simulink library "AEMS_Standard_Library"  (R2016b)
settings: Solver=ode45  StartTime=0.0  StopTime=10.0  RelTol=1e-3
undefined symbols (not defined in the file or in its folder): BkPY, carto, Cbx_extegr, Cbx_lpegrsys, Cbx_portegr, Cnx_bnk_nr_conf, Cnx_cyl_nr_conf, ConfigManagement, configuration_management, Cxx_dcm_io_tmr_end_xxxx, Cxx_dcm_rt_tmr_end, Cxx_DID_xxxx_IO_max, Cxx_DID_xxxx_IO_min, Cxx_egrhsofs, Cxx_vmaniegi, DEM_DEBOUNCE_FREEZE, DEM_DTR_CTL_INVISIBLE, DEM_DTR_CTL_NORMAL, Dem_DtrId2_XXX, Dem_DtrId3_XXX, Dem_DtrId4_XXX, Dem_DtrId5_XXX, Dem_DtrId6_XXX, Dem_DtrId7_XXX, Dem_DtrId8_XXX, Dem_DtrId9_XXX, Dem_DtrId_XXX, Dem_EnableConditionId2_XXX, Dem_EnableConditionId3_XXX, Dem_EnableConditionId4_XXX, Dem_EnableConditionId5_XXX, Dem_EnableConditionId6_XXX, Dem_EnableConditionId7_XXX, Dem_EnableConditionId8_XXX, Dem_EnableConditionId_XXX, Dem_EventId, Dem_EventId2_XXX, Dem_EventId3_XXX, Dem_EventId4_XXX, Dem_EventId5_XXX, Dem_EventId6_XXX, Dem_EventId7_XXX, Dem_EventId8_XXX, Dem_EventId9_XXX, Dem_EventId_Device_Faulttype, Dem_EventId_XXX, DEM_IUMPR_GENERAL_DENOMINATOR, DEM_OPCYC_IGNITION, Dem_RatioId2_XXX, Dem_RatioId3_XXX, Dem_RatioId4_XXX, Dem_RatioId5_XXX, Dem_RatioId6_XXX, Dem_RatioId7_XXX, Dem_RatioId8_XXX, Dem_RatioId_XXX, Dem_StorageConditionId2_XXX, Dem_StorageConditionId3_XXX, Dem_StorageConditionId4_XXX, Dem_StorageConditionId5_XXX ... (+65)
libraries: AEMS_Standard_Library x477, simulink x2
(part 3 of 39)

== system AEMS_Standard_Library/DCM ==
  note: AUTOSAR INTERFACE for DCM TO BE USED IN
      | DataServices or RoutineServices_DIDAbstract_AUTOSAR_Interface
  note: Applicative DCM:
      | To be used in functional specifications
  note: Supplier API Call:
      | To be used to call Supplier API
  AEMS_API_SUPPLIER_CALL : Subsystem  Tag=[LIB]  mask(AEMS_API_SUPPLIER_CALL){portName=port, operationPrototype=API_Supplier_Fcn(IN uint8 In1[12], IN int16 In2[3], OUT single Out1[1]), NumInputs=2, NumOutputs=1, API_Name=Ex_API, Ptr_Arg=01}
      mask prompts: portName "Client Port name"; operationPrototype "API Supplier Function Call Name"; NumInputs "Number of Inputs"; NumOutputs "Number of Outputs"; Ptr_Arg "Pointer_Arguments"
      mask help:
      | This block is used to call the function prototype specified as "Supplier_API_name" in the generated C-code with
      | arguments provided as inputs.
      |
      | Example Supplier API Call:
      | API_Supplier_Fcn(IN uint8 In1[12], IN int16 In2[3], OUT single Out1[1]);
      |
      | Code expected:
      | API_Supplier_Fcn(In1,In2,&Out1)
      mask init:
      | BlkName = gcb;
      | hblk = gcbh;
      | 
      | % if strcmp(get_param(hblk,'LinkStatus'),'resolved')
      | %     set_param(hblk,'LinkStatus','inactive');
      | % else
      | %     %already disabled or none
      | % end
      | datatypelist={'uint8','int8','uint16','int16','uint32','int32','boolean','single','double'};
      | 
      | ProtoTypeStr = get_param(hblk,'operationPrototype');
      | 
      | % try 
      | flag_err = 0;
      | st = regexp(ProtoTypeStr,'(');
      | et = regexp(ProtoTypeStr,')');
      | if isempty(st) || isempty(et)
      |     flag_err = 1;
      |     error('OperationPrototype must contain braces ''('' and '')''');
      | elseif length(st)>1 || length(et)>1
      |     flag_err = 1;
      |     error('Invalid format for  Operation Prototype');
      | else
      |     API_Name = ProtoTypeStr(1:(st-1));
      |     Proto_str = regexprep(ProtoTypeStr,[API_Name,'|',')|('],'');
      |     
      |     %     Proto_str = regexprep(regexprep(ProtoTypeStr,API_Name,''),')|(',''); % alternative
      |     
      |     NumInputs = length(regexp(ProtoTypeStr,'IN |INOUT '));
      |     NumOutputs = length(regexp(ProtoTypeStr,'[^IN]OUT '));
      |     
      |     if NumInputs ~= 0 || NumOutputs ~= 0
      |         parts= regexp(strtrim(regexp(strtrim(Proto_str),',','split')),' ' ,'split');
      |     else
      |         parts ='';
      |     end
      |     for i=1:numel(parts)
      |         if numel(parts{i})~=3
      |             flag_err = 1;
      |             error('Invalid format:Avoid extra spaces in between Argument literals (Ex: IN single In1)');
      |         end
      |     end
      | end
      | 
      | inporthdl = find_system(BlkName,'FollowLinks','on','LookunderMasks','all','regexp','on','BlockType','Inport');
      | outporthdl = find_system(BlkName,'FollowLinks','on','LookunderMasks','all','regexp','on','BlockType','Outport');
      | 
      | isChanged=0; 
      | for i=1:numel(parts) 
      |     if ~isempty(regexp(parts{i}{1},'IN|OUT|INOUT','once'))
      |         if ismember(parts{i}{2},datatypelist) || isempty(parts{i}{2})
      |             tmp_DT = parts{i}{2};
      |         else
      |             error(['Datatype ''' parts{i}{2} ''' is invalid']);
      |         end
      |         if length(regexp(parts{i}{3},'['))==1 && length(regexp(parts{i}{3},']'))==1
      |             % dimension specified
      |         elseif isempty(regexp(parts{i}{3},'[')) && isempty(regexp(parts{i}{3},']'))
      |             % dimension not specified
      |         else
      |             error('Avoid Extra/unexpected braces (''['' and '']'').Enter Correct Format(Ex IN uint8 a[12])');
      |         end
      |         [Port_name,Port_Dim] = strtok(parts{i}{3},'[');
      |         if ~isempty(regexp(Port_name,'^\d|^_','once'))
      |             error(sprintf(['Invalid Inport/Outport name:' Port_name '\nName should start with an alphabet']));
      |         elseif ~isempty(regexp(Port_name,'_$','once'))
      |             error(sprintf(['Invalid Inport/Outport name:' Port_name '\nName shouldn''t end with underscore(_)']));
      |         else
      | 
      |             if isempty(regexp(Port_Dim,'([\d+\])','once'))
      |                 error('Incorrect Dimension entered.Check and Enter Correct Format(Ex IN uint8 a[12])');
      |             else
      |                 tmp_Dim = strtok(Port_Dim,'^[]$');
      |             end
      | 
      |             if isempty(regexp(Port_name,'\W','once'))
      |                 tmp_Name = Port_name;
      |             else
      |                 error('Special characters otherthan underscore( _ ) are not allowed in Port names');
      |             end
      |         end
      |     end
      |     if strcmp(parts{i}{1},'IN') || strcmp(parts{i}{1},'INOUT')
      |         %         NumInputs = NumInputs+1;
      |         In_InOut_Names = tmp_Name;
      |         In_InOut_Types = tmp_DT;
      |         In_InOut_Dim = tmp_Dim;
      |         inporthdl = find_system(hblk,'FollowLinks','on','LookunderMasks','all','regexp','on','BlockType','Inport','Name',In_InOut_Names);
      |         if isempty(inporthdl)
      |            isChanged=1; 
      |            break;
      |         else
      |            datatype=get_param(inporthdl,'OutDataTypeStr'); 
      |            indim=get_param(inporthdl,'PortDimensions');
      |            if ~isequal(datatype,In_InOut_Types)||~isequal(indim,In_InOut_Dim)
      |               isChanged=1; 
      |               break;               
      |            end
      |         end
      |     elseif strcmp(parts{i}{1},'OUT')
      |         %         NumOutputs = NumOutputs+1;
      |         Out_Names = tmp_Name;
      |         Out_Types = tmp_DT;
      |         Out_Dim = tmp_Dim;
      |         outporthdl = find_system(hblk,'FollowLinks','on','LookunderMasks','all','regexp','on','BlockType','Outport','Name',Out_Names);
      |         if isempty(outporthdl)
      |            isChanged=1; 
      |            break;
      |         else
      |            datatype=get_param(outporthdl,'OutDataTypeStr'); 
      |            indim=get_param(outporthdl,'PortDimensions');
      |            if ~isequal(datatype,Out_Types)||~isequal(indim,Out_Dim)
      |               isChanged=1; 
      |               break;               
      |            end
      |         end        
      |         
      |     else
      |         error('Direction must be IN, INOUT or OUT');
      |     end
      | end      
      | % if length(st)~=length(et) && flag_err_occur==0
      | %     flag_err = 1;
      | %     errordlg('Invalid format for  Operation Prototype');
      | % end
      | 
      | % if evalin('base','flag_err')==0
      | if flag_err == 0&&isChanged
      |     % To Remove Lines and Terminator/Ground
      |     lines = find_system(hblk,'LookUnderMasks','all','FollowLinks','On','FindAll','on','Type','line');
      |     GndTer = find_system(hblk,'LookUnderMasks','all','FollowLinks','On','regexp','On','FindAll','on','BlockType','^Ground$|^Terminator$|^DataTypeConversion$');
      | %     GndTer = find_system(hblk,'LookUnderMasks','all','FollowLinks','On','regexp','On','FindAll','on','BlockType','^Ground$|^Terminator$');
      |     tobe_del = [lines;GndTer];
      |     for i=1:length(tobe_del)
      |         try
      |             delete_line(tobe_del(i));
      |         catch
      |             delete_block(tobe_del(i));
      |         end
      |     end
      |     
      |     In_InOut_Names = {};
      |     In_InOut_Types = {};
      |     In_InOut_Dim = {};
      |     Out_Names = {};
      |     Out_Types = {};
      |     Out_Dim = {};
      |     % NumOutputs = 0;
      |     % NumInputs = 0;
      |     % parts = evalin('base','parts');
      |     for i=1:numel(parts)
      |         if ~isempty(regexp(parts{i}{1},'IN|OUT|INOUT','once'))
      |             if ismember(parts{i}{2},datatypelist) || isempty(parts{i}{2})
      |                 tmp_DT = parts{i}{2};
      |             else
      |                 error(['Datatype ''' parts{i}{2} ''' is invalid']);
      |             end
      |             if length(regexp(parts{i}{3},'['))==1 && length(regexp(parts{i}{3},']'))==1
      |                 % dimension specified
      |             elseif isempty(regexp(parts{i}{3},'[')) && isempty(regexp(parts{i}{3},']'))
      |                 % dimension not specified
      |             else
      |                 error('Avoid Extra/unexpected braces (''['' and '']'').Enter Correct Format(Ex IN uint8 a[12])');
      |             end
      |             [Port_name,Port_Dim] = strtok(parts{i}{3},'[');
      |             if ~isempty(regexp(Port_name,'^\d|^_','once'))
      |                 error(sprintf(['Invalid Inport/Outport name:' Port_name '\nName should start with an alphabet']));
      |             elseif ~isempty(regexp(Port_name,'_$','once'))
      |                 error(sprintf(['Invalid Inport/Outport name:' Port_name '\nName shouldn''t end with underscore(_)']));
      |             else
      |                 
      |                 if isempty(regexp(Port_Dim,'([\d+\])','once'))
      |                     error('Incorrect Dimension entered.Check and Enter Correct Format(Ex IN uint8 a[12])');
      |                 else
      |                     tmp_Dim = strtok(Port_Dim,'^[]$');
      |                 end
      |                 
      |                 if isempty(regexp(Port_name,'\W','once'))
      |                     tmp_Name = Port_name;
      |                 else
      |                     error('Special characters otherthan underscore( _ ) are not allowed in Port names');
      |                 end
      |             end
      |         end
      |         if strcmp(parts{i}{1},'IN') || strcmp(parts{i}{1},'INOUT')
      |             %         NumInputs = NumInputs+1;
      |             In_InOut_Names = [In_InOut_Names,tmp_Name];
      |             In_InOut_Types = [In_InOut_Types,tmp_DT];
      |             In_InOut_Dim = [In_InOut_Dim,tmp_Dim];
      |         elseif strcmp(parts{i}{1},'OUT')
      |             %         NumOutputs = NumOutputs+1;
      |             Out_Names = [Out_Names,tmp_Name];
      |             Out_Types = [Out_Types,tmp_DT];
      |             Out_Dim = [Out_Dim,tmp_Dim];
      |         else
      |             error('Direction must be IN, INOUT or OUT');
      |         end
      |     end
      |     
      |     %To delete unwanted Inport/Outport blocks
      |     Inports_exist = get_param(find_system(BlkName,'LookUnderMasks','All','FollowLinks','On','regexp','On','BlockType','Inport'),'Name');
      |     Outports_exist = get_param(find_system(BlkName,'LookUnderMasks','All','FollowLinks','On','regexp','On','BlockType','Outport'),'Name');
      |     Inports_to_be_del = setdiff(Inports_exist,In_InOut_Names);
      |     Outports_to_be_del = setdiff(Outports_exist,Out_Names);
      |     ports_to_be_del = [Inports_to_be_del;Outports_to_be_del];
      |     for n=1:numel(ports_to_be_del)
      |         delete_block([BlkName,'/',ports_to_be_del{n}]);
      |     end
      |     
      |     tmp_in_out_names = [In_InOut_Names,Out_Names];
      |     
      |     if ~isequal(length(unique(tmp_in_out_names)),length(tmp_in_out_names))
      |         error('Port names must be unique')
      |     else
      |         %To add In Ports
      |         % NumInputs = numel(IN_OR_INOUT_Strings);
      |         for n=1:NumInputs
      |             Pos_Y1 = (10+((n-1)*40));
      |             Blk_Pos = [20,Pos_Y1,50,Pos_Y1+15];
      |             Term_Pos = [115,Pos_Y1,135,Pos_Y1+20];
      |             try
      |                 add_block('built-in/Inport',[BlkName,'/',In_InOut_Names{n}]);
      |             catch
      |                 set_param([BlkName,'/',In_InOut_Names{n}],'Port',num2str(n));
      |             end
      |             set_param([BlkName,'/',In_InOut_Names{n}],...
      |                 'Position',Blk_Pos,...
      |                 'OutDataTypeStr',In_InOut_Types{n},...
      |                 'PortDimensions',In_InOut_Dim{n},...
      |                 'Backgroundcolor','green');
      |             add_block('built-in/Terminator',[BlkName,'/T_',In_InOut_Names{n}],'Position',Term_Pos,'ShowName','off');
      |             add_line(BlkName,[In_InOut_Names{n},'/1'],['T_',In_InOut_Names{n},'/1']);
      |         end
      |         
      |         %To add Out Ports
      |         for n=1:NumOutputs
      |             Pos_Y1 = (10+((n-1)*40));
      |             Blk_Pos = [400,Pos_Y1,430,Pos_Y1+15];
      |             Con_Pos = [300,Pos_Y1,330,Pos_Y1+20];
      |             Gnd_Pos = [210,Pos_Y1,230,Pos_Y1+20];
      |             try
      |                 add_block('built-in/Outport',[BlkName,'/',Out_Names{n}],'Position',Blk_Pos,'OutDataTypeStr',Out_Types{n},'Backgroundcolor','orange');
      |             catch
      |                 set_param([BlkName,'/',Out_Names{n}],'Port',num2str(n),'Position',Blk_Pos,'OutDataTypeStr',Out_Types{n},'Backgroundcolor','orange');
      |             end
      |             set_param([BlkName,'/',Out_Names{n}],...
      |                 'Position',Blk_Pos,...
      |                 'OutDataTypeStr',Out_Types{n},...
      |                 'PortDimensions',Out_Dim{n},...
      |                 'Backgroundcolor','orange');
      |             add_block('built-in/Ground',[BlkName,'/G_',Out_Names{n}],'Position',Gnd_Pos,'ShowName','off');
      |             add_block('built-in/DatatypeConversion',[BlkName,'/Conv_',Out_Names{n}],'Position',Con_Pos,'ShowName','off');
      |             add_line(BlkName,['Conv_',Out_Names{n},'/1'],[Out_Names{n},'/1']);
      |             add_line(BlkName,['G_',Out_Names{n},'/1'],['Conv_',Out_Names{n},'/1']);
      |         end
      |         mask_data = Simulink.Mask.get(hblk);
      |         mask_data.IconOpaque = 'off';
      |         set_param(hblk,...
      |             'NumInputs',num2str(NumInputs),...
      |             'NumOutputs',num2str(NumOutputs));
      |     end
      | end
      | 
      | % catch ErrorException
      | %     Message = sprintf('Message : %s', ErrorException.message);
      | %     for ie=1:length(ErrorException.stack)
      | %         Message = sprintf('%s\nFilename : %s', Message, ErrorException.stack(ie).file);
      | %         Message = sprintf('%s\nName : %s', Message, ErrorException.stack(ie).name);
      | %         Message = sprintf('%s\nLine : %i', Message, ErrorException.stack(ie).line);
      | %     end
      | %     disp(Message);    
      | % end
      settings: AttributesFormatString="%<MaskType>\\nPrototype: %<operationPrototype>\\nNo. of Inputs :%<NumInputs>  No of Outputs: %<NumOutputs>"
      mask Display: disp('AEMS_API_SUPPLIER_CALL');
  AEMS_APP_DID_WRITEDATA : Subsystem  Tag=[LIB]  mask(AEMS_APP_DID_WRITEDATA){}
      mask help:
      | Gets the output for DID variable depends on request write from tools. If Request write comes from DCM tools, DID variable get value from DCM tools if not it gets value from strategy’s calculation.
      |
      | -INPUTS-
      | Value_DID_Write: DID value from DCM Tools
      | Request_Write_DID: Request Write from DCM Tools
      | Strategy: Value calculated from strategy
      |
      | -OUTPUTS-
      | DID_Var: Value DID for output
      settings: AttributesFormatString=%<MaskType>
      mask Help:
      | eval('path_lib=fileparts(which(''AEMS_Standard_Library''));');
      | mskblk=get_param(gcbh,'MaskType');
      | doc_path = [path_lib '\Help\',mskblk,'.pdf'];
      | eval('open(doc_path)');
  AEMS_APP_REQUEST_IOCONTROL : Subsystem  Tag=[LIB]  mask(AEMS_APP_REQUEST_IOCONTROL){DIDAbstract=DCM_IO_XXXX, Cxx_dcm_io_tmr_end_xxxx=Cxx_dcm_io_tmr_end_xxxx}
      mask prompts: DIDAbstract "DID Abstract"; Cxx_dcm_io_tmr_end_xxxx "Duration of Timer (in milisecond)"
      mask help:
      | IO request is activated by Request from ShortTermAdjustment under the control of
      | Request from ReturnControlToECU status, Generic Condition, Specific condition and Timer End of XXXX DID Abstract.
      | Output value of DID XXXX from Callback ShorttermAdjustment.
      |
      | -INPUTS-
      | Req_stadj_stt_xxxx: Request from ShortTermAdjustment status of XXXX
      | Req_rcecu_stt_xxxx: Request from ReturnControlToECU status of XXXX
      | Generic_Condition: Generic condition
      | Specific_Condition_xxxx: Specific condition of XXXX DID
      | Value_Write_stadj_xxxx: Value of IO Signal DID XXX from ShortTermAdjustment
      |
      | -OUTPUTS-
      | Flag_io_request_xxxx: Output of IO request controlled
      | Flag_dcm_io_tmr_end_xxxx: Timer End Status of XXXX
      | Dcm_io_tmr_xxxx: Timer which counts down from value defined in Duration of Timer in miliseconde
      | Val_io_request_xxxx: Output of IO Signal DID XXX from ShortTermAdjustment
      |
      | -PARAMETERS-
      | DID Abstract: Abstract of DID
      | Duration of Timer: Duration of Timer
      mask init:
      | hh = gcbh;
      | DIDAbstractstr=get_param(hh,'DIDAbstract'); 
      | namepi1=strcat('Req_stadj_',DIDAbstractstr);
      | namepi2=strcat('Req_rcecu_',DIDAbstractstr);
      | namepi3='Generic_Condition';
      | namepi4=strcat('Specific_Condition_',DIDAbstractstr);
      | namepi5=strcat('Value_Write_stadj_',DIDAbstractstr);
      | % namepi5='Req_tmr_end_xxxx';
      | namepo1=strcat('Flag_io_request_',DIDAbstractstr);
      | namepo2=strcat('Flag_dcm_io_tmr_end_',DIDAbstractstr);
      | namepo3=strcat('Dcm_io_tmr_',DIDAbstractstr);
      | namepo4=strcat('Val_io_request_',DIDAbstractstr);
      | 
      | % encond_b1 = find_system(gcb,'LookUnderMasks','all','FollowLinks','on','Name','Cxx_dcm_io_tmr_end_xxxx');
      | % set_param([encond_b1{:}],'Value',char(Cxx_dcm_io_tmr_end_xxxx));
      settings: AttributesFormatString=|
      | %<MaskType>
      | DID Abstract : %<DIDAbstract>
      | Duration of Timer : %<Cxx_dcm_io_tmr_end_xxxx>
      mask Help:
      | eval('path_lib=fileparts(which(''AEMS_Standard_Library''));');
      | mskblk=get_param(gcbh,'MaskType');
      | doc_path = [path_lib '\Help\',mskblk,'.pdf'];
      | eval('open(doc_path)');
      mask Display:
      | port_label('input',1,namepi1);
      | port_label('input',2,namepi2);
      | port_label('input',3,namepi3);
      | port_label('input',4,namepi4);
      | port_label('input',5,namepi5);
      | port_label('output',1,namepo1);
      | port_label('output',2,namepo2);
      | port_label('output',3,namepo3);
      | port_label('output',4,namepo4);
  AEMS_APP_REQUEST_ROUTINE : Subsystem  Tag=[LIB]  mask(AEMS_APP_REQUEST_ROUTINE){DIDAbstract=DCM_RT_XXXX, Cxx_dcm_rt_tmr_end=Cxx_dcm_rt_tmr_end}
      mask prompts: DIDAbstract "RID Abstract"; Cxx_dcm_rt_tmr_end "Duration of Timer (in second)"
      mask help:
      | Retrun flags of START Callback STOP Callback from DCM.
      | Flag START is enabled if there is a change from Request of START Callback
      | Flag STOP is activated by Request from STOP Callback, Generic Condition, Specific condition and Timer End of XXXX RID Abstract.
      |
      | -INPUTS-
      | Req_sta_stt_xxxx: Request from START status of XXXX
      | Req_stop_stt_xxxx: Request from STOP status of XXXX
      | Generic_Condition: Generic condition
      | Specific_Condition_xxxx: Specific condition of XXXX RID during Routine Callback
      |
      | -OUTPUTS-
      | Flag_sta_xxxx: Output of request from START Callback
      | Flag_stop_xxxx: Output of request from STOP Callback
      | Flag_dcm_rt_tmr_end: Timer End Status
      | Dcm_rt_tmr_xxxx: Timer which counts down from value defined in Duration of Timer in seconde
      |
      | -PARAMETERS-
      | RID Abstract: Abstract of RID
      | Duration of Timer: Duration of Timer
      mask init:
      | hh = gcbh;
      | DIDAbstractstr=get_param(hh,'DIDAbstract'); 
      | namepi1=strcat('Req_sta_',DIDAbstractstr);
      | namepi2=strcat('Req_stop_',DIDAbstractstr);
      | namepi3='Generic_Condition';
      | namepi4=strcat('Specific_Condition_',DIDAbstractstr);
      | % namepi5='Req_tmr_end';
      | namepo1=strcat('Flag_sta_',DIDAbstractstr);
      | namepo2=strcat('Flag_stop_',DIDAbstractstr);
      | namepo3=strcat('Flag_dcm_rt_tmr_end_',DIDAbstractstr);
      | namepo4=strcat('Dcm_rt_tmr_',DIDAbstractstr);
      settings: AttributesFormatString=|
      | %<MaskType>
      | RID Abstract : %<DIDAbstract>
      | Duration of Timer : %<Cxx_dcm_rt_tmr_end>
      mask Help:
      | eval('path_lib=fileparts(which(''AEMS_Standard_Library''));');
      | mskblk=get_param(gcbh,'MaskType');
      | doc_path = [path_lib '\Help\',mskblk,'.pdf'];
      | eval('open(doc_path)');
      mask Display:
      | port_label('input',1,namepi1);
      | port_label('input',2,namepi2);
      | port_label('input',3,namepi3);
      | port_label('input',4,namepi4);
      | port_label('output',1,namepo1);
      | port_label('output',2,namepo2);
      | port_label('output',3,namepo3);
      | port_label('output',4,namepo4);
  AEMS_DCM_CLEARDIAGNOSTICINFORMATION : Subsystem  Tag=[LIB]  mask(AEMS_DCM_CLEARDIAGNOSTICINFORMATION){}
      mask help:
      | This library calls AUTOSAR standard functions.
      | To know more details, please refer AUTOSAR [SWS_Dem_00241].
      settings: AttributesFormatString=%<MaskType>
      mask Display: disp(['Dcm_ClearDiagnosticInformation']);
  AEMS_DCM_CONDITIONCHECKREAD : Subsystem  Tag=[LIB]  mask(AEMS_DCM_CONDITIONCHECKREAD){DIDAbstract=DCM_DID_XXXX}
      mask prompts: DIDAbstract "DID Abstract"
      mask help:
      | This function requests to the application to start the execution of a routine.
      | AUTOSAR Interface: Xxx_Start (Ref. [SWS_Dcm_01203])
      |
      | Std_ReturnType Xxx_ConditionCheckRead(Dcm_NegativeResponseCodeType* ErrorCode)
      |
      | ErrorCode: terminated to represent return values to DCM Tools.
      |
      | -INPUTS-
      | Condition_checkread: Condition check read
      |
      | -PARAMETERS-
      | DID Abstract: Abstract of DID
      mask init:
      | hh = gcbh;
      | DIDAbstractstr=get_param(hh,'DIDAbstract'); 
      | Callbkstr=strcat('DataServices_',strtrim(DIDAbstractstr),'_WriteData');
      | namepi1='Generic_Conditions_Routine';
      | namepi2=strcat('Specific_Conditions_Routine_',DIDAbstractstr);
      | namepi3='Routine_Status';
      | namepi4=strcat('Routine_Status_',DIDAbstractstr);
      | namepo1=strcat('Flag_Request_',DIDAbstractstr);
      settings: AttributesFormatString=|
      | %<MaskType>
      | DID Abstract: %<DIDAbstract>
      mask Help:
      | eval('path_lib=fileparts(which(''AEMS_Standard_Library''));');
      | mskblk=get_param(gcbh,'MaskType');
      | doc_path = [path_lib '\Help\',mskblk,'.pdf'];
      | eval('open(doc_path)');
      mask Display:
      | % port_label('input',1,namepi1);
      | % port_label('input',2,namepi2);
      | % port_label('input',3,namepi3);
      | % port_label('input',4,namepi4);
      | % port_label('output',1,namepo1);
  AEMS_DCM_DID_READDATA : Subsystem  Tag=[LIB]  mask(AEMS_DCM_DID_READDATA){DIDAbstract=DCM_DID_XXXX, NumDIDVar=1, RaDIDVar1=[0,255], OffsetDIDVar1=0, ResolDIDVar1=1, DataTypeDIDVar1=uint8, In_DID_Name_1=Val_did_1, RaDIDVar2=[-128,127], OffsetDIDVar2=0, ResolDIDVar2=1, DataTypeDIDVar2=int8, In_DID_Name_2=Val_did_2, RaDIDVar3=[0,1], OffsetDIDVar3=0, ResolDIDVar3=1, DataTypeDIDVar3=int16, In_DID_Name_3=Val_did_3, RaDIDVar4=[0,100], OffsetDIDVar4=0, ResolDIDVar4=1, DataTypeDIDVar4=uint8, In_DID_Name_4=Val_did_4, RaDIDVar5=[0,1], OffsetDIDVar5=0, ResolDIDVar5=1, DataTypeDIDVar5=uint16, In_DID_Name_5=Val_did_5, RaDIDVar6=[0,1], OffsetDIDVar6=0, ResolDIDVar6=1, DataTypeDIDVar6=uint8, In_DID_Name_6=Val_did_6, RaDIDVar7=[0,1], OffsetDIDVar7=0, ResolDIDVar7=1, DataTypeDIDVar7=uint8, In_DID_Name_7=Val_did_7, RaDIDVar8=[0,1], OffsetDIDVar8=0, ResolDIDVar8=1, DataTypeDIDVar8=uint8, In_DID_Name_8=Val_did_8, RaDIDVar9=[0,1], OffsetDIDVar9=0, ResolDIDVar9=1, DataTypeDIDVar9=uint8, In_DID_Name_9=Val_did_9, RaDIDVar10=[0,1], OffsetDIDVar10=0, ResolDIDVar10=1, DataTypeDIDVar10=uint8, In_DID_Name_10=Val_did_10, RaDIDVar11=[0,1], OffsetDIDVar11=0, ResolDIDVar11=1, DataTypeDIDVar11=uint8, In_DID_Name_11=Val_did_11, RaDIDVar12=[0,1], OffsetDIDVar12=0, ResolDIDVar12=1, DataTypeDIDVar12=uint8, In_DID_Name_12=Val_did_12, RaDIDVar13=[0,1], OffsetDIDVar13=0, ResolDIDVar13=1, DataTypeDIDVar13=uint8, In_DID_Name_13=Val_did_13, RaDIDVar14=[0,1], OffsetDIDVar14=0, ResolDIDVar14=1, DataTypeDIDVar14=uint8, In_DID_Name_14=Val_did_14, RaDIDVar15=[0,1], OffsetDIDVar15=0, ResolDIDVar15=1, DataTypeDIDVar15=uint8, In_DID_Name_15=Val_did_15, RaDIDVar16=[0,1], OffsetDIDVar16=0, ResolDIDVar16=1, DataTypeDIDVar16=uint8, In_DID_Name_16=Val_did_16, RaDIDVar17=[0,1], OffsetDIDVar17=0, ResolDIDVar17=1, DataTypeDIDVar17=uint8, In_DID_Name_17=Val_did_17, RaDIDVar18=[0,1], OffsetDIDVar18=0, ResolDIDVar18=1, DataTypeDIDVar18=uint8, In_DID_Name_18=Val_did_18, RaDIDVar19=[0,1], OffsetDIDVar19=0, ResolDIDVar19=1, DataTypeDIDVar19=uint8, In_DID_Name_19=Val_did_19, RaDIDVar20=[0,1], OffsetDIDVar20=0, ResolDIDVar20=1, DataTypeDIDVar20=uint8, In_DID_Name_20=Val_did_20, RaDIDVar21=[0,1], OffsetDIDVar21=0, ResolDIDVar21=1, DataTypeDIDVar21=uint8, In_DID_Name_21=Val_did_21, RaDIDVar22=[0,1], OffsetDIDVar22=0, ResolDIDVar22=1, DataTypeDIDVar22=uint8, In_DID_Name_22=Val_did_22, RaDIDVar23=[0,1], OffsetDIDVar23=0, ResolDIDVar23=1, DataTypeDIDVar23=uint8, In_DID_Name_23=Val_did_23, RaDIDVar24=[0,1], OffsetDIDVar24=0, ResolDIDVar24=1, DataTypeDIDVar24=uint8, In_DID_Name_24=Val_did_24, RaDIDVar25=[0,1], OffsetDIDVar25=0, ResolDIDVar25=1, DataTypeDIDVar25=uint8, In_DID_Name_25=Val_did_25, RaDIDVar26=[0,1], OffsetDIDVar26=0, ResolDIDVar26=1, DataTypeDIDVar26=uint8, In_DID_Name_26=Val_did_26, RaDIDVar27=[0,1], OffsetDIDVar27=0, ResolDIDVar27=1, DataTypeDIDVar27=uint8, In_DID_Name_27=Val_did_27, RaDIDVar28=[0,1], OffsetDIDVar28=0, ResolDIDVar28=1, DataTypeDIDVar28=uint8, In_DID_Name_28=Val_did_28, RaDIDVar29=[0,1], OffsetDIDVar29=0, ResolDIDVar29=1, DataTypeDIDVar29=uint8, In_DID_Name_29=Val_did_29, RaDIDVar30=[0,1], OffsetDIDVar30=0, ResolDIDVar30=1, DataTypeDIDVar30=uint8, In_DID_Name_30=Val_did_30, RaDIDVar31=[0,1], OffsetDIDVar31=0, ResolDIDVar31=1, DataTypeDIDVar31=uint8, In_DID_Name_31=Val_did_31, RaDIDVar32=[0,1], OffsetDIDVar32=0, ResolDIDVar32=1, DataTypeDIDVar32=uint8, In_DID_Name_32=Val_did_32, RaDIDVar33=[0,1], OffsetDIDVar33=0, ResolDIDVar33=1, DataTypeDIDVar33=uint8, In_DID_Name_33=Val_did_33, RaDIDVar34=[0,1], OffsetDIDVar34=0, ResolDIDVar34=1, DataTypeDIDVar34=uint8, In_DID_Name_34=Val_did_34, RaDIDVar35=[0,1], OffsetDIDVar35=0, ResolDIDVar35=1, DataTypeDIDVar35=uint8, In_DID_Name_35=Val_did_35, RaDIDVar36=[0,1], OffsetDIDVar36=0, ResolDIDVar36=1, DataTypeDIDVar36=uint8, In_DID_Name_36=Val_did_36, RaDIDVar37=[0,1], OffsetDIDVar37=0, ResolDIDVar37=1, DataTypeDIDVar37=uint8, In_DID_Name_37=Val_did_37, RaDIDVar38=[0,1], OffsetDIDVar38=0, ResolDIDVar38=1, DataTypeDIDVar38=uint8, In_DID_Name_38=Val_did_38, RaDIDVar39=[0,1], OffsetDIDVar39=0, ResolDIDVar39=1, DataTypeDIDVar39=uint8, In_DID_Name_39=Val_did_39, RaDIDVar40=[0,1], OffsetDIDVar40=0, ResolDIDVar40=1, DataTypeDIDVar40=uint8, In_DID_Name_40=Val_did_40, RaDIDVar41=[0,1], OffsetDIDVar41=0, ResolDIDVar41=1, DataTypeDIDVar41=uint8, In_DID_Name_41=Val_did_41, RaDIDVar42=[0,1], OffsetDIDVar42=0, ResolDIDVar42=1, DataTypeDIDVar42=uint8, In_DID_Name_42=Val_did_42, RaDIDVar43=[0,1], OffsetDIDVar43=0, ResolDIDVar43=1, DataTypeDIDVar43=uint8, In_DID_Name_43=Val_did_43, RaDIDVar44=[0,1], OffsetDIDVar44=0, ResolDIDVar44=1, DataTypeDIDVar44=uint8, In_DID_Name_44=Val_did_44, RaDIDVar45=[0,1], OffsetDIDVar45=0, ResolDIDVar45=1, DataTypeDIDVar45=uint8, In_DID_Name_45=Val_did_45, RaDIDVar46=[0,1], OffsetDIDVar46=0, ResolDIDVar46=1, DataTypeDIDVar46=uint8, In_DID_Name_46=Val_did_46, RaDIDVar47=[0,1], OffsetDIDVar47=0, ResolDIDVar47=1, DataTypeDIDVar47=uint8, In_DID_Name_47=Val_did_47, RaDIDVar48=[0,1], OffsetDIDVar48=0, ResolDIDVar48=1, DataTypeDIDVar48=uint8, In_DID_Name_48=Val_did_48, RaDIDVar49=[0,1], OffsetDIDVar49=0, ResolDIDVar49=1, DataTypeDIDVar49=uint8, In_DID_Name_49=Val_did_49, RaDIDVar50=[0,1], OffsetDIDVar50=0, ResolDIDVar50=1, DataTypeDIDVar50=uint8, In_DID_Name_50=Val_did_50, RaDIDVar51=[0,1], OffsetDIDVar51=0, ResolDIDVar51=1, DataTypeDIDVar51=uint8, In_DID_Name_51=Val_did_51, RaDIDVar52=[0,1], OffsetDIDVar52=0, ResolDIDVar52=1, DataTypeDIDVar52=uint8, In_DID_Name_52=Val_did_52, RaDIDVar53=[0,1], OffsetDIDVar53=0, ResolDIDVar53=1, DataTypeDIDVar53=uint8, In_DID_Name_53=Val_did_53, RaDIDVar54=[0,1], OffsetDIDVar54=0, ResolDIDVar54=1, DataTypeDIDVar54=uint8, In_DID_Name_54=Val_did_54, RaDIDVar55=[0,1], OffsetDIDVar55=0, ResolDIDVar55=1, DataTypeDIDVar55=uint8, In_DID_Name_55=Val_did_55, RaDIDVar56=[0,1], OffsetDIDVar56=0, ResolDIDVar56=1, DataTypeDIDVar56=uint8, In_DID_Name_56=Val_did_56, RaDIDVar57=[0,1], OffsetDIDVar57=0, ResolDIDVar57=1, DataTypeDIDVar57=uint8, In_DID_Name_57=Val_did_57, RaDIDVar58=[0,1], OffsetDIDVar58=0, ResolDIDVar58=1, DataTypeDIDVar58=uint8, In_DID_Name_58=Val_did_58, RaDIDVar59=[0,1], OffsetDIDVar59=0, ResolDIDVar59=1, DataTypeDIDVar59=uint8, In_DID_Name_59=Val_did_59, RaDIDVar60=[0,1], OffsetDIDVar60=0, ResolDIDVar60=1, DataTypeDIDVar60=uint8, In_DID_Name_60=Val_did_60, RaDIDVar61=[0,1], OffsetDIDVar61=0, ResolDIDVar61=1, DataTypeDIDVar61=uint8, In_DID_Name_61=Val_did_61, RaDIDVar62=[0,1], OffsetDIDVar62=0, ResolDIDVar62=1, DataTypeDIDVar62=uint8, In_DID_Name_62=Val_did_62, RaDIDVar63=[0,1], OffsetDIDVar63=0, ResolDIDVar63=1, DataTypeDIDVar63=uint8, In_DID_Name_63=Val_did_63, RaDIDVar64=[0,1], OffsetDIDVar64=0, ResolDIDVar64=1, DataTypeDIDVar64=uint8, In_DID_Name_64=Val_did_64, RaDIDVar65=[0,1], OffsetDIDVar65=0, ResolDIDVar65=1, DataTypeDIDVar65=uint8, In_DID_Name_65=Val_did_65, RaDIDVar66=[0,1], OffsetDIDVar66=0, ResolDIDVar66=1, DataTypeDIDVar66=uint8, In_DID_Name_66=Val_did_66, RaDIDVar67=[0,1], OffsetDIDVar67=0, ResolDIDVar67=1, DataTypeDIDVar67=uint8, In_DID_Name_67=Val_did_67, RaDIDVar68=[0,1], OffsetDIDVar68=0, ResolDIDVar68=1, DataTypeDIDVar68=uint8, In_DID_Name_68=Val_did_68, RaDIDVar69=[0,1], OffsetDIDVar69=0, ResolDIDVar69=1, DataTypeDIDVar69=uint8, In_DID_Name_69=Val_did_69, RaDIDVar70=[0,1], OffsetDIDVar70=0, ResolDIDVar70=1, DataTypeDIDVar70=uint8, In_DID_Name_70=Val_did_70, RaDIDVar71=[0,1], OffsetDIDVar71=0, ResolDIDVar71=1, DataTypeDIDVar71=uint8, In_DID_Name_71=Val_did_71, RaDIDVar72=[0,1], OffsetDIDVar72=0, ResolDIDVar72=1, DataTypeDIDVar72=uint8, In_DID_Name_72=Val_did_72, RaDIDVar73=[0,1], OffsetDIDVar73=0, ResolDIDVar73=1, DataTypeDIDVar73=uint8, In_DID_Name_73=Val_did_73, RaDIDVar74=[0,1], OffsetDIDVar74=0, ResolDIDVar74=1, DataTypeDIDVar74=uint8, In_DID_Name_74=Val_did_74, RaDIDVar75=[0,1], OffsetDIDVar75=0, ResolDIDVar75=1, DataTypeDIDVar75=uint8, In_DID_Name_75=Val_did_75, RaDIDVar76=[0,1], OffsetDIDVar76=0, ResolDIDVar76=1, DataTypeDIDVar76=uint8, In_DID_Name_76=Val_did_76, RaDIDVar77=[0,1], OffsetDIDVar77=0, ResolDIDVar77=1, DataTypeDIDVar77=uint8, In_DID_Name_77=Val_did_77, RaDIDVar78=[0,1], OffsetDIDVar78=0, ResolDIDVar78=1, DataTypeDIDVar78=uint8, In_DID_Name_78=Val_did_78, RaDIDVar79=[0,1], OffsetDIDVar79=0, ResolDIDVar79=1, DataTypeDIDVar79=uint8, In_DID_Name_79=Val_did_79, RaDIDVar80=[0,1], OffsetDIDVar80=0, ResolDIDVar80=1, DataTypeDIDVar80=uint8, In_DID_Name_80=Val_did_80, RaDIDVar81=[0,1], OffsetDIDVar81=0, ResolDIDVar81=1, DataTypeDIDVar81=uint8, In_DID_Name_81=Val_did_81, RaDIDVar82=[0,1], OffsetDIDVar82=0, ResolDIDVar82=1, DataTypeDIDVar82=uint8, In_DID_Name_82=Val_did_82, RaDIDVar83=[0,1], OffsetDIDVar83=0, ResolDIDVar83=1, DataTypeDIDVar83=uint8, In_DID_Name_83=Val_did_83, RaDIDVar84=[0,1], OffsetDIDVar84=0, ResolDIDVar84=1, DataTypeDIDVar84=uint8, In_DID_Name_84=Val_did_84, RaDIDVar85=[0,1], OffsetDIDVar85=0, ResolDIDVar85=1, DataTypeDIDVar85=uint8, In_DID_Name_85=Val_did_85, RaDIDVar86=[0,1], OffsetDIDVar86=0, ResolDIDVar86=1, DataTypeDIDVar86=uint8, In_DID_Name_86=Val_did_86, RaDIDVar87=[0,1], OffsetDIDVar87=0, ResolDIDVar87=1, DataTypeDIDVar87=uint8, In_DID_Name_87=Val_did_87, RaDIDVar88=[0,1], OffsetDIDVar88=0, ResolDIDVar88=1, DataTypeDIDVar88=uint8, In_DID_Name_88=Val_did_88, RaDIDVar89=[0,1], OffsetDIDVar89=0, ResolDIDVar89=1, DataTypeDIDVar89=uint8, In_DID_Name_89=Val_did_89, RaDIDVar90=[0,1], OffsetDIDVar90=0, ResolDIDVar90=1, DataTypeDIDVar90=uint8, In_DID_Name_90=Val_did_90, RaDIDVar91=[0,1], OffsetDIDVar91=0, ResolDIDVar91=1, DataTypeDIDVar91=uint8, In_DID_Name_91=Val_did_91, RaDIDVar92=[0,1], OffsetDIDVar92=0, ResolDIDVar92=1, DataTypeDIDVar92=uint8, In_DID_Name_92=Val_did_92, RaDIDVar93=[0,1], OffsetDIDVar93=0, ResolDIDVar93=1, DataTypeDIDVar93=uint8, In_DID_Name_93=Val_did_93, RaDIDVar94=[0,1], OffsetDIDVar94=0, ResolDIDVar94=1, DataTypeDIDVar94=uint8, In_DID_Name_94=Val_did_94, RaDIDVar95=[0,1], OffsetDIDVar95=0, ResolDIDVar95=1, DataTypeDIDVar95=uint8, In_DID_Name_95=Val_did_95, RaDIDVar96=[0,1], OffsetDIDVar96=0, ResolDIDVar96=1, DataTypeDIDVar96=uint8, In_DID_Name_96=Val_did_96, RaDIDVar97=[0,1], OffsetDIDVar97=0, ResolDIDVar97=1, DataTypeDIDVar97=uint8, In_DID_Name_97=Val_did_97, RaDIDVar98=[0,1], OffsetDIDVar98=0, ResolDIDVar98=1, DataTypeDIDVar98=uint8, In_DID_Name_98=Val_did_98, RaDIDVar99=[0,1], OffsetDIDVar99=0, ResolDIDVar99=1, DataTypeDIDVar99=uint8, In_DID_Name_99=Val_did_99, RaDIDVar100=[0,1], OffsetDIDVar100=0, ResolDIDVar100=1, DataTypeDIDVar100=uint8, In_DID_Name_100=Val_did_100, RaDIDVar101=[0,1], OffsetDIDVar101=0, ResolDIDVar101=1, DataTypeDIDVar101=uint8, In_DID_Name_101=Val_did_101, RaDIDVar102=[0,1], OffsetDIDVar102=0, ResolDIDVar102=1, DataTypeDIDVar102=uint8, In_DID_Name_102=Val_did_102, RaDIDVar103=[0,1], OffsetDIDVar103=0, ResolDIDVar103=1, DataTypeDIDVar103=uint8, In_DID_Name_103=Val_did_103, RaDIDVar104=[0,1], OffsetDIDVar104=0, ResolDIDVar104=1, DataTypeDIDVar104=uint8, In_DID_Name_104=Val_did_104, RaDIDVar105=[0,1], OffsetDIDVar105=0, ResolDIDVar105=1, DataTypeDIDVar105=uint8, In_DID_Name_105=Val_did_105, RaDIDVar106=[0,1], OffsetDIDVar106=0, ResolDIDVar106=1, DataTypeDIDVar106=uint8, In_DID_Name_106=Val_did_106, RaDIDVar107=[0,1], OffsetDIDVar107=0, ResolDIDVar107=1, DataTypeDIDVar107=uint8, In_DID_Name_107=Val_did_107, RaDIDVar108=[0,1], OffsetDIDVar108=0, ResolDIDVar108=1, DataTypeDIDVar108=uint8, In_DID_Name_108=Val_did_108, RaDIDVar109=[0,1], OffsetDIDVar109=0, ResolDIDVar109=1, DataTypeDIDVar109=uint8, In_DID_Name_109=Val_did_109, RaDIDVar110=[0,1], OffsetDIDVar110=0, ResolDIDVar110=1, DataTypeDIDVar110=uint8, In_DID_Name_110=Val_did_110, RaDIDVar111=[0,1], OffsetDIDVar111=0, ResolDIDVar111=1, DataTypeDIDVar111=uint8, In_DID_Name_111=Val_did_111, RaDIDVar112=[0,1], OffsetDIDVar112=0, ResolDIDVar112=1, DataTypeDIDVar112=uint8, In_DID_Name_112=Val_did_112, RaDIDVar113=[0,1], OffsetDIDVar113=0, ResolDIDVar113=1, DataTypeDIDVar113=uint8, In_DID_Name_113=Val_did_113, RaDIDVar114=[0,1], OffsetDIDVar114=0, ResolDIDVar114=1, DataTypeDIDVar114=uint8, In_DID_Name_114=Val_did_114, RaDIDVar115=[0,1], OffsetDIDVar115=0, ResolDIDVar115=1, DataTypeDIDVar115=uint8, In_DID_Name_115=Val_did_115, RaDIDVar116=[0,1], OffsetDIDVar116=0, ResolDIDVar116=1, DataTypeDIDVar116=uint8, In_DID_Name_116=Val_did_116, RaDIDVar117=[0,1], OffsetDIDVar117=0, ResolDIDVar117=1, DataTypeDIDVar117=uint8, In_DID_Name_117=Val_did_117, RaDIDVar118=[0,1], OffsetDIDVar118=0, ResolDIDVar118=1, DataTypeDIDVar118=uint8, In_DID_Name_118=Val_did_118, RaDIDVar119=[0,1], OffsetDIDVar119=0, ResolDIDVar119=1, DataTypeDIDVar119=uint8, In_DID_Name_119=Val_did_119, RaDIDVar120=[0,1], OffsetDIDVar120=0, ResolDIDVar120=1, DataTypeDIDVar120=uint8, In_DID_Name_120=Val_did_120, RaDIDVar121=[0,1], OffsetDIDVar121=0, ResolDIDVar121=1, DataTypeDIDVar121=uint8, In_DID_Name_121=Val_did_121, RaDIDVar122=[0,1], OffsetDIDVar122=0, ResolDIDVar122=1, DataTypeDIDVar122=uint8, In_DID_Name_122=Val_did_122, RaDIDVar123=[0,1], OffsetDIDVar123=0, ResolDIDVar123=1, DataTypeDIDVar123=uint8, In_DID_Name_123=Val_did_123, RaDIDVar124=[0,1], OffsetDIDVar124=0, ResolDIDVar124=1, DataTypeDIDVar124=uint8, In_DID_Name_124=Val_did_124, RaDIDVar125=[0,1], OffsetDIDVar125=0, ResolDIDVar125=1, DataTypeDIDVar125=uint8, In_DID_Name_125=Val_did_125, RaDIDVar126=[0,1], OffsetDIDVar126=0, ResolDIDVar126=1, DataTypeDIDVar126=uint8, In_DID_Name_126=Val_did_126, RaDIDVar127=[0,1], OffsetDIDVar127=0, ResolDIDVar127=1, DataTypeDIDVar127=uint8, In_DID_Name_127=Val_did_127, RaDIDVar128=[0,1], OffsetDIDVar128=0, ResolDIDVar128=1, DataTypeDIDVar128=uint8, In_DID_Name_128=Val_did_128, RaDIDVar129=[0,1], OffsetDIDVar129=0, ResolDIDVar129=1, DataTypeDIDVar129=uint8, In_DID_Name_129=Val_did_129, RaDIDVar130=[0,1], OffsetDIDVar130=0, ResolDIDVar130=1, DataTypeDIDVar130=uint8, In_DID_Name_130=Val_did_130, RaDIDVar131=[0,1], OffsetDIDVar131=0, ResolDIDVar131=1, DataTypeDIDVar131=uint8, In_DID_Name_131=Val_did_131, RaDIDVar132=[0,1], OffsetDIDVar132=0, ResolDIDVar132=1, DataTypeDIDVar132=uint8, In_DID_Name_132=Val_did_132, RaDIDVar133=[0,1], OffsetDIDVar133=0, ResolDIDVar133=1, DataTypeDIDVar133=uint8, In_DID_Name_133=Val_did_133, RaDIDVar134=[0,1], OffsetDIDVar134=0, ResolDIDVar134=1, DataTypeDIDVar134=uint8, In_DID_Name_134=Val_did_134, RaDIDVar135=[0,1], OffsetDIDVar135=0, ResolDIDVar135=1, DataTypeDIDVar135=uint8, In_DID_Name_135=Val_did_135, RaDIDVar136=[0,1], OffsetDIDVar136=0, ResolDIDVar136=1, DataTypeDIDVar136=uint8, In_DID_Name_136=Val_did_136, RaDIDVar137=[0,1], OffsetDIDVar137=0, ResolDIDVar137=1, DataTypeDIDVar137=uint8, In_DID_Name_137=Val_did_137, RaDIDVar138=[0,1], OffsetDIDVar138=0, ResolDIDVar138=1, DataTypeDIDVar138=uint8, In_DID_Name_138=Val_did_138, RaDIDVar139=[0,1], OffsetDIDVar139=0, ResolDIDVar139=1, DataTypeDIDVar139=uint8, In_DID_Name_139=Val_did_139, RaDIDVar140=[0,1], OffsetDIDVar140=0, ResolDIDVar140=1, DataTypeDIDVar140=uint8, In_DID_Name_140=Val_did_140, RaDIDVar141=[0,1], OffsetDIDVar141=0, ResolDIDVar141=1, DataTypeDIDVar141=uint8, In_DID_Name_141=Val_did_141, RaDIDVar142=[0,1], OffsetDIDVar142=0, ResolDIDVar142=1, DataTypeDIDVar142=uint8, In_DID_Name_142=Val_did_142, RaDIDVar143=[0,1], OffsetDIDVar143=0, ResolDIDVar143=1, DataTypeDIDVar143=uint8, In_DID_Name_143=Val_did_143, RaDIDVar144=[0,1], OffsetDIDVar144=0, ResolDIDVar144=1, DataTypeDIDVar144=uint8, In_DID_Name_144=Val_did_144, RaDIDVar145=[0,1], OffsetDIDVar145=0, ResolDIDVar145=1, DataTypeDIDVar145=uint8, In_DID_Name_145=Val_did_145, RaDIDVar146=[0,1], OffsetDIDVar146=0, ResolDIDVar146=1, DataTypeDIDVar146=uint8, In_DID_Name_146=Val_did_146, RaDIDVar147=[0,1], OffsetDIDVar147=0, ResolDIDVar147=1, DataTypeDIDVar147=uint8, In_DID_Name_147=Val_did_147, RaDIDVar148=[0,1], OffsetDIDVar148=0, ResolDIDVar148=1, DataTypeDIDVar148=uint8, In_DID_Name_148=Val_did_148, RaDIDVar149=[0,1], OffsetDIDVar149=0, ResolDIDVar149=1, DataTypeDIDVar149=uint8, In_DID_Name_149=Val_did_149, RaDIDVar150=[0,1], OffsetDIDVar150=0, ResolDIDVar150=1, DataTypeDIDVar150=uint8, In_DID_Name_150=Val_did_150, RaDIDVar151=[0,1], OffsetDIDVar151=0, ResolDIDVar151=1, DataTypeDIDVar151=uint8, In_DID_Name_151=Val_did_151, RaDIDVar152=[0,1], OffsetDIDVar152=0, ResolDIDVar152=1, DataTypeDIDVar152=uint8, In_DID_Name_152=Val_did_152, RaDIDVar153=[0,1], OffsetDIDVar153=0, ResolDIDVar153=1, DataTypeDIDVar153=uint8, In_DID_Name_153=Val_did_153, RaDIDVar154=[0,1], OffsetDIDVar154=0, ResolDIDVar154=1, DataTypeDIDVar154=uint8, In_DID_Name_154=Val_did_154, RaDIDVar155=[0,1], OffsetDIDVar155=0, ResolDIDVar155=1, DataTypeDIDVar155=uint8, In_DID_Name_155=Val_did_155, RaDIDVar156=[0,1], OffsetDIDVar156=0, ResolDIDVar156=1, DataTypeDIDVar156=uint8, In_DID_Name_156=Val_did_156, RaDIDVar157=[0,1], OffsetDIDVar157=0, ResolDIDVar157=1, DataTypeDIDVar157=uint8, In_DID_Name_157=Val_did_157, RaDIDVar158=[0,1], OffsetDIDVar158=0, ResolDIDVar158=1, DataTypeDIDVar158=uint8, In_DID_Name_158=Val_did_158, RaDIDVar159=[0,1], OffsetDIDVar159=0, ResolDIDVar159=1, DataTypeDIDVar159=uint8, In_DID_Name_159=Val_did_159, RaDIDVar160=[0,1], OffsetDIDVar160=0, ResolDIDVar160=1, DataTypeDIDVar160=uint8, In_DID_Name_160=Val_did_160, RaDIDVar161=[0,1], OffsetDIDVar161=0, ResolDIDVar161=1, DataTypeDIDVar161=uint8, In_DID_Name_161=Val_did_161, RaDIDVar162=[0,1], OffsetDIDVar162=0, ResolDIDVar162=1, DataTypeDIDVar162=uint8, In_DID_Name_162=Val_did_162, RaDIDVar163=[0,1], OffsetDIDVar163=0, ResolDIDVar163=1, DataTypeDIDVar163=uint8, In_DID_Name_163=Val_did_163, RaDIDVar164=[0,1], OffsetDIDVar164=0, ResolDIDVar164=1, DataTypeDIDVar164=uint8, In_DID_Name_164=Val_did_164, RaDIDVar165=[0,1], OffsetDIDVar165=0, ResolDIDVar165=1, DataTypeDIDVar165=uint8, In_DID_Name_165=Val_did_165, RaDIDVar166=[0,1], OffsetDIDVar166=0, ResolDIDVar166=1, DataTypeDIDVar166=uint8, In_DID_Name_166=Val_did_166, RaDIDVar167=[0,1], OffsetDIDVar167=0, ResolDIDVar167=1, DataTypeDIDVar167=uint8, In_DID_Name_167=Val_did_167, RaDIDVar168=[0,1], OffsetDIDVar168=0, ResolDIDVar168=1, DataTypeDIDVar168=uint8, In_DID_Name_168=Val_did_168, RaDIDVar169=[0,1], OffsetDIDVar169=0, ResolDIDVar169=1, DataTypeDIDVar169=uint8, In_DID_Name_169=Val_did_169, RaDIDVar170=[0,1], OffsetDIDVar170=0, ResolDIDVar170=1, DataTypeDIDVar170=uint8, In_DID_Name_170=Val_did_170, RaDIDVar171=[0,1], OffsetDIDVar171=0, ResolDIDVar171=1, DataTypeDIDVar171=uint8, In_DID_Name_171=Val_did_171, RaDIDVar172=[0,1], OffsetDIDVar172=0, ResolDIDVar172=1, DataTypeDIDVar172=uint8, In_DID_Name_172=Val_did_172, RaDIDVar173=[0,1], OffsetDIDVar173=0, ResolDIDVar173=1, DataTypeDIDVar173=uint8, In_DID_Name_173=Val_did_173, RaDIDVar174=[0,1], OffsetDIDVar174=0, ResolDIDVar174=1, DataTypeDIDVar174=uint8, In_DID_Name_174=Val_did_174, RaDIDVar175=[0,1], OffsetDIDVar175=0, ResolDIDVar175=1, DataTypeDIDVar175=uint8, In_DID_Name_175=Val_did_175, RaDIDVar176=[0,1], OffsetDIDVar176=0, ResolDIDVar176=1, DataTypeDIDVar176=uint8, In_DID_Name_176=Val_did_176, RaDIDVar177=[0,1], OffsetDIDVar177=0, ResolDIDVar177=1, DataTypeDIDVar177=uint8, In_DID_Name_177=Val_did_177, RaDIDVar178=[0,1], OffsetDIDVar178=0, ResolDIDVar178=1, DataTypeDIDVar178=uint8, In_DID_Name_178=Val_did_178, RaDIDVar179=[0,1], OffsetDIDVar179=0, ResolDIDVar179=1, DataTypeDIDVar179=uint8, In_DID_Name_179=Val_did_179, RaDIDVar180=[0,1], OffsetDIDVar180=0, ResolDIDVar180=1, DataTypeDIDVar180=uint8, In_DID_Name_180=Val_did_180, RaDIDVar181=[0,1], OffsetDIDVar181=0, ResolDIDVar181=1, DataTypeDIDVar181=uint8, In_DID_Name_181=Val_did_181, RaDIDVar182=[0,1], OffsetDIDVar182=0, ResolDIDVar182=1, DataTypeDIDVar182=uint8, In_DID_Name_182=Val_did_182, RaDIDVar183=[0,1], OffsetDIDVar183=0, ResolDIDVar183=1, DataTypeDIDVar183=uint8, In_DID_Name_183=Val_did_183, RaDIDVar184=[0,1], OffsetDIDVar184=0, ResolDIDVar184=1, DataTypeDIDVar184=uint8, In_DID_Name_184=Val_did_184, RaDIDVar185=[0,1], OffsetDIDVar185=0, ResolDIDVar185=1, DataTypeDIDVar185=uint8, In_DID_Name_185=Val_did_185, RaDIDVar186=[0,1], OffsetDIDVar186=0, ResolDIDVar186=1, DataTypeDIDVar186=uint8, In_DID_Name_186=Val_did_186, RaDIDVar187=[0,1], OffsetDIDVar187=0, ResolDIDVar187=1, DataTypeDIDVar187=uint8, In_DID_Name_187=Val_did_187, RaDIDVar188=[0,1], OffsetDIDVar188=0, ResolDIDVar188=1, DataTypeDIDVar188=uint8, In_DID_Name_188=Val_did_188, RaDIDVar189=[0,1], OffsetDIDVar189=0, ResolDIDVar189=1, DataTypeDIDVar189=uint8, In_DID_Name_189=Val_did_189, RaDIDVar190=[0,1], OffsetDIDVar190=0, ResolDIDVar190=1, DataTypeDIDVar190=uint8, In_DID_Name_190=Val_did_190, RaDIDVar191=[0,1], OffsetDIDVar191=0, ResolDIDVar191=1, DataTypeDIDVar191=uint8, In_DID_Name_191=Val_did_191, RaDIDVar192=[0,1], OffsetDIDVar192=0, ResolDIDVar192=1, DataTypeDIDVar192=uint8, In_DID_Name_192=Val_did_192, RaDIDVar193=[0,1], OffsetDIDVar193=0, ResolDIDVar193=1, DataTypeDIDVar193=uint8, In_DID_Name_193=Val_did_193, RaDIDVar194=[0,1], OffsetDIDVar194=0, ResolDIDVar194=1, DataTypeDIDVar194=uint8, In_DID_Name_194=Val_did_194, RaDIDVar195=[0,1], OffsetDIDVar195=0, ResolDIDVar195=1, DataTypeDIDVar195=uint8, In_DID_Name_195=Val_did_195, RaDIDVar196=[0,1], OffsetDIDVar196=0, ResolDIDVar196=1, DataTypeDIDVar196=uint8, In_DID_Name_196=Val_did_196, RaDIDVar197=[0,1], OffsetDIDVar197=0, ResolDIDVar197=1, DataTypeDIDVar197=uint8, In_DID_Name_197=Val_did_197, RaDIDVar198=[0,1], OffsetDIDVar198=0, ResolDIDVar198=1, DataTypeDIDVar198=uint8, In_DID_Name_198=Val_did_198, RaDIDVar199=[0,1], OffsetDIDVar199=0, ResolDIDVar199=1, DataTypeDIDVar199=uint8, In_DID_Name_199=Val_did_199, RaDIDVar200=[0,1], OffsetDIDVar200=0, ResolDIDVar200=1, DataTypeDIDVar200=uint8, In_DID_Name_200=Val_did_200, RaDIDVar201=[0,1], OffsetDIDVar201=0, ResolDIDVar201=1, DataTypeDIDVar201=uint8, In_DID_Name_201=Val_did_201, RaDIDVar202=[0,1], OffsetDIDVar202=0, ResolDIDVar202=1, DataTypeDIDVar202=uint8, In_DID_Name_202=Val_did_202, RaDIDVar203=[0,1], OffsetDIDVar203=0, ResolDIDVar203=1, DataTypeDIDVar203=uint8, In_DID_Name_203=Val_did_203, RaDIDVar204=[0,1], OffsetDIDVar204=0, ResolDIDVar204=1, DataTypeDIDVar204=uint8, In_DID_Name_204=Val_did_204, RaDIDVar205=[0,1], OffsetDIDVar205=0, ResolDIDVar205=1, DataTypeDIDVar205=uint8, In_DID_Name_205=Val_did_205, RaDIDVar206=[0,1], OffsetDIDVar206=0, ResolDIDVar206=1, DataTypeDIDVar206=uint8, In_DID_Name_206=Val_did_206, RaDIDVar207=[0,1], OffsetDIDVar207=0, ResolDIDVar207=1, DataTypeDIDVar207=uint8, In_DID_Name_207=Val_did_207, RaDIDVar208=[0,1], OffsetDIDVar208=0, ResolDIDVar208=1, DataTypeDIDVar208=uint8, In_DID_Name_208=Val_did_208, RaDIDVar209=[0,1], OffsetDIDVar209=0, ResolDIDVar209=1, DataTypeDIDVar209=uint8, In_DID_Name_209=Val_did_209, RaDIDVar210=[0,1], OffsetDIDVar210=0, ResolDIDVar210=1, DataTypeDIDVar210=uint8, In_DID_Name_210=Val_did_210, RaDIDVar211=[0,1], OffsetDIDVar211=0, ResolDIDVar211=1, DataTypeDIDVar211=uint8, In_DID_Name_211=Val_did_211, RaDIDVar212=[0,1], OffsetDIDVar212=0, ResolDIDVar212=1, DataTypeDIDVar212=uint8, In_DID_Name_212=Val_did_212, RaDIDVar213=[0,1], OffsetDIDVar213=0, ResolDIDVar213=1, DataTypeDIDVar213=uint8, In_DID_Name_213=Val_did_213, RaDIDVar214=[0,1], OffsetDIDVar214=0, ResolDIDVar214=1, DataTypeDIDVar214=uint8, In_DID_Name_214=Val_did_214, RaDIDVar215=[0,1], OffsetDIDVar215=0, ResolDIDVar215=1, DataTypeDIDVar215=uint8, In_DID_Name_215=Val_did_215, RaDIDVar216=[0,1], OffsetDIDVar216=0, ResolDIDVar216=1, DataTypeDIDVar216=uint8, In_DID_Name_216=Val_did_216, RaDIDVar217=[0,1], OffsetDIDVar217=0, ResolDIDVar217=1, DataTypeDIDVar217=uint8, In_DID_Name_217=Val_did_217, RaDIDVar218=[0,1], OffsetDIDVar218=0, ResolDIDVar218=1, DataTypeDIDVar218=uint8, In_DID_Name_218=Val_did_218, RaDIDVar219=[0,1], OffsetDIDVar219=0, ResolDIDVar219=1, DataTypeDIDVar219=uint8, In_DID_Name_219=Val_did_219, RaDIDVar220=[0,1], OffsetDIDVar220=0, ResolDIDVar220=1, DataTypeDIDVar220=uint8, In_DID_Name_220=Val_did_220, RaDIDVar221=[0,1], OffsetDIDVar221=0, ResolDIDVar221=1, DataTypeDIDVar221=uint8, In_DID_Name_221=Val_did_221, RaDIDVar222=[0,1], OffsetDIDVar222=0, ResolDIDVar222=1, DataTypeDIDVar222=uint8, In_DID_Name_222=Val_did_222, RaDIDVar223=[0,1], OffsetDIDVar223=0, ResolDIDVar223=1, DataTypeDIDVar223=uint8, In_DID_Name_223=Val_did_223, RaDIDVar224=[0,1], OffsetDIDVar224=0, ResolDIDVar224=1, DataTypeDIDVar224=uint8, In_DID_Name_224=Val_did_224, RaDIDVar225=[0,1], OffsetDIDVar225=0, ResolDIDVar225=1, DataTypeDIDVar225=uint8, In_DID_Name_225=Val_did_225, RaDIDVar226=[0,1], OffsetDIDVar226=0, ResolDIDVar226=1, DataTypeDIDVar226=uint8, In_DID_Name_226=Val_did_226, RaDIDVar227=[0,1], OffsetDIDVar227=0, ResolDIDVar227=1, DataTypeDIDVar227=uint8, In_DID_Name_227=Val_did_227, RaDIDVar228=[0,1], OffsetDIDVar228=0, ResolDIDVar228=1, DataTypeDIDVar228=uint8, In_DID_Name_228=Val_did_228, RaDIDVar229=[0,1], OffsetDIDVar229=0, ResolDIDVar229=1, DataTypeDIDVar229=uint8, In_DID_Name_229=Val_did_229, RaDIDVar230=[0,1], OffsetDIDVar230=0, ResolDIDVar230=1, DataTypeDIDVar230=uint8, In_DID_Name_230=Val_did_230, RaDIDVar231=[0,1], OffsetDIDVar231=0, ResolDIDVar231=1, DataTypeDIDVar231=uint8, In_DID_Name_231=Val_did_231, RaDIDVar232=[0,1], OffsetDIDVar232=0, ResolDIDVar232=1, DataTypeDIDVar232=uint8, In_DID_Name_232=Val_did_232, RaDIDVar233=[0,1], OffsetDIDVar233=0, ResolDIDVar233=1, DataTypeDIDVar233=uint8, In_DID_Name_233=Val_did_233, RaDIDVar234=[0,1], OffsetDIDVar234=0, ResolDIDVar234=1, DataTypeDIDVar234=uint8, In_DID_Name_234=Val_did_234, RaDIDVar235=[0,1], OffsetDIDVar235=0, ResolDIDVar235=1, DataTypeDIDVar235=uint8, In_DID_Name_235=Val_did_235, RaDIDVar236=[0,1], OffsetDIDVar236=0, ResolDIDVar236=1, DataTypeDIDVar236=uint8, In_DID_Name_236=Val_did_236, RaDIDVar237=[0,1], OffsetDIDVar237=0, ResolDIDVar237=1, DataTypeDIDVar237=uint8, In_DID_Name_237=Val_did_237, RaDIDVar238=[0,1], OffsetDIDVar238=0, ResolDIDVar238=1, DataTypeDIDVar238=uint8, In_DID_Name_238=Val_did_238, RaDIDVar239=[0,1], OffsetDIDVar239=0, ResolDIDVar239=1, DataTypeDIDVar239=uint8, In_DID_Name_239=Val_did_239, RaDIDVar240=[0,1], OffsetDIDVar240=0, ResolDIDVar240=1, DataTypeDIDVar240=uint8, In_DID_Name_240=Val_did_240, RaDIDVar241=[0,1], OffsetDIDVar241=0, ResolDIDVar241=1, DataTypeDIDVar241=uint8, In_DID_Name_241=Val_did_241, RaDIDVar242=[0,1], OffsetDIDVar242=0, ResolDIDVar242=1, DataTypeDIDVar242=uint8, In_DID_Name_242=Val_did_242, RaDIDVar243=[0,1], OffsetDIDVar243=0, ResolDIDVar243=1, DataTypeDIDVar243=uint8, In_DID_Name_243=Val_did_243, RaDIDVar244=[0,1], OffsetDIDVar244=0, ResolDIDVar244=1, DataTypeDIDVar244=uint8, In_DID_Name_244=Val_did_244, RaDIDVar245=[0,1], OffsetDIDVar245=0, ResolDIDVar245=1, DataTypeDIDVar245=uint8, In_DID_Name_245=Val_did_245, RaDIDVar246=[0,1], OffsetDIDVar246=0, ResolDIDVar246=1, DataTypeDIDVar246=uint8, In_DID_Name_246=Val_did_246, RaDIDVar247=[0,1], OffsetDIDVar247=0, ResolDIDVar247=1, DataTypeDIDVar247=uint8, In_DID_Name_247=Val_did_247, RaDIDVar248=[0,1], OffsetDIDVar248=0, ResolDIDVar248=1, DataTypeDIDVar248=uint8, In_DID_Name_248=Val_did_248, RaDIDVar249=[0,1], OffsetDIDVar249=0, ResolDIDVar249=1, DataTypeDIDVar249=uint8, In_DID_Name_249=Val_did_249, RaDIDVar250=[0,1], OffsetDIDVar250=0, ResolDIDVar250=1, DataTypeDIDVar250=uint8, In_DID_Name_250=Val_did_250, RaDIDVar251=[0,1], OffsetDIDVar251=0, ResolDIDVar251=1, DataTypeDIDVar251=uint8, In_DID_Name_251=Val_did_251, RaDIDVar252=[0,1], OffsetDIDVar252=0, ResolDIDVar252=1, DataTypeDIDVar252=uint8, In_DID_Name_252=Val_did_252, RaDIDVar253=[0,1], OffsetDIDVar253=0, ResolDIDVar253=1, DataTypeDIDVar253=uint8, In_DID_Name_253=Val_did_253, RaDIDVar254=[0,1], OffsetDIDVar254=0, ResolDIDVar254=1, DataTypeDIDVar254=uint8, In_DID_Name_254=Val_did_254, RaDIDVar255=[0,1], OffsetDIDVar255=0, ResolDIDVar255=1, DataTypeDIDVar255=uint8, In_DID_Name_255=Val_did_255, RaDIDVar256=[0,1], OffsetDIDVar256=0, ResolDIDVar256=1, DataTypeDIDVar256=uint8, In_DID_Name_256=Val_did_256, RaDIDVar257=[0,1], OffsetDIDVar257=0, ResolDIDVar257=1, DataTypeDIDVar257=uint8, In_DID_Name_257=Val_did_257, RaDIDVar258=[0,1], OffsetDIDVar258=0, ResolDIDVar258=1, DataTypeDIDVar258=uint8, In_DID_Name_258=Val_did_258, RaDIDVar259=[0,1], OffsetDIDVar259=0, ResolDIDVar259=1, DataTypeDIDVar259=uint8, In_DID_Name_259=Val_did_259, RaDIDVar260=[0,1], OffsetDIDVar260=0, ResolDIDVar260=1, DataTypeDIDVar260=uint8, In_DID_Name_260=Val_did_260, RaDIDVar261=[0,1], OffsetDIDVar261=0, ResolDIDVar261=1, DataTypeDIDVar261=uint8, In_DID_Name_261=Val_did_261, RaDIDVar262=[0,1], OffsetDIDVar262=0, ResolDIDVar262=1, DataTypeDIDVar262=uint8, In_DID_Name_262=Val_did_262, RaDIDVar263=[0,1], OffsetDIDVar263=0, ResolDIDVar263=1, DataTypeDIDVar263=uint8, In_DID_Name_263=Val_did_263, RaDIDVar264=[0,1], OffsetDIDVar264=0, ResolDIDVar264=1, DataTypeDIDVar264=uint8, In_DID_Name_264=Val_did_264, RaDIDVar265=[0,1], OffsetDIDVar265=0, ResolDIDVar265=1, DataTypeDIDVar265=uint8, In_DID_Name_265=Val_did_265, RaDIDVar266=[0,1], OffsetDIDVar266=0, ResolDIDVar266=1, DataTypeDIDVar266=uint8, In_DID_Name_266=Val_did_266, RaDIDVar267=[0,1], OffsetDIDVar267=0, ResolDIDVar267=1, DataTypeDIDVar267=uint8, In_DID_Name_267=Val_did_267, RaDIDVar268=[0,1], OffsetDIDVar268=0, ResolDIDVar268=1, DataTypeDIDVar268=uint8, In_DID_Name_268=Val_did_268, RaDIDVar269=[0,1], OffsetDIDVar269=0, ResolDIDVar269=1, DataTypeDIDVar269=uint8, In_DID_Name_269=Val_did_269, RaDIDVar270=[0,1], OffsetDIDVar270=0, ResolDIDVar270=1, DataTypeDIDVar270=uint8, In_DID_Name_270=Val_did_270, RaDIDVar271=[0,1], OffsetDIDVar271=0, ResolDIDVar271=1, DataTypeDIDVar271=uint8, In_DID_Name_271=Val_did_271, RaDIDVar272=[0,1], OffsetDIDVar272=0, ResolDIDVar272=1, DataTypeDIDVar272=uint8, In_DID_Name_272=Val_did_272, RaDIDVar273=[0,1], OffsetDIDVar273=0, ResolDIDVar273=1, DataTypeDIDVar273=uint8, In_DID_Name_273=Val_did_273, RaDIDVar274=[0,1], OffsetDIDVar274=0, ResolDIDVar274=1, DataTypeDIDVar274=uint8, In_DID_Name_274=Val_did_274, RaDIDVar275=[0,1], OffsetDIDVar275=0, ResolDIDVar275=1, DataTypeDIDVar275=uint8, In_DID_Name_275=Val_did_275, RaDIDVar276=[0,1], OffsetDIDVar276=0, ResolDIDVar276=1, DataTypeDIDVar276=uint8, In_DID_Name_276=Val_did_276, RaDIDVar277=[0,1], OffsetDIDVar277=0, ResolDIDVar277=1, DataTypeDIDVar277=uint8, In_DID_Name_277=Val_did_277, RaDIDVar278=[0,1], OffsetDIDVar278=0, ResolDIDVar278=1, DataTypeDIDVar278=uint8, In_DID_Name_278=Val_did_278, RaDIDVar279=[0,1], OffsetDIDVar279=0, ResolDIDVar279=1, DataTypeDIDVar279=uint8, In_DID_Name_279=Val_did_279, RaDIDVar280=[0,1], OffsetDIDVar280=0, ResolDIDVar280=1, DataTypeDIDVar280=uint8, In_DID_Name_280=Val_did_280, RaDIDVar281=[0,1], OffsetDIDVar281=0, ResolDIDVar281=1, DataTypeDIDVar281=uint8, In_DID_Name_281=Val_did_281, RaDIDVar282=[0,1], OffsetDIDVar282=0, ResolDIDVar282=1, DataTypeDIDVar282=uint8, In_DID_Name_282=Val_did_282, RaDIDVar283=[0,1], OffsetDIDVar283=0, ResolDIDVar283=1, DataTypeDIDVar283=uint8, In_DID_Name_283=Val_did_283, RaDIDVar284=[0,1], OffsetDIDVar284=0, ResolDIDVar284=1, DataTypeDIDVar284=uint8, In_DID_Name_284=Val_did_284, RaDIDVar285=[0,1], OffsetDIDVar285=0, ResolDIDVar285=1, DataTypeDIDVar285=uint8, In_DID_Name_285=Val_did_285, RaDIDVar286=[0,1], OffsetDIDVar286=0, ResolDIDVar286=1, DataTypeDIDVar286=uint8, In_DID_Name_286=Val_did_286, RaDIDVar287=[0,1], OffsetDIDVar287=0, ResolDIDVar287=1, DataTypeDIDVar287=uint8, In_DID_Name_287=Val_did_287, RaDIDVar288=[0,1], OffsetDIDVar288=0, ResolDIDVar288=1, DataTypeDIDVar288=uint8, In_DID_Name_288=Val_did_288, RaDIDVar289=[0,1], OffsetDIDVar289=0, ResolDIDVar289=1, DataTypeDIDVar289=uint8, In_DID_Name_289=Val_did_289, RaDIDVar290=[0,1], OffsetDIDVar290=0, ResolDIDVar290=1, DataTypeDIDVar290=uint8, In_DID_Name_290=Val_did_290, RaDIDVar291=[0,1], OffsetDIDVar291=0, ResolDIDVar291=1, DataTypeDIDVar291=uint8, In_DID_Name_291=Val_did_291, RaDIDVar292=[0,1], OffsetDIDVar292=0, ResolDIDVar292=1, DataTypeDIDVar292=uint8, In_DID_Name_292=Val_did_292, RaDIDVar293=[0,1], OffsetDIDVar293=0, ResolDIDVar293=1, DataTypeDIDVar293=uint8, In_DID_Name_293=Val_did_293, RaDIDVar294=[0,1], OffsetDIDVar294=0, ResolDIDVar294=1, DataTypeDIDVar294=uint8, In_DID_Name_294=Val_did_294, RaDIDVar295=[0,1], OffsetDIDVar295=0, ResolDIDVar295=1, DataTypeDIDVar295=uint8, In_DID_Name_295=Val_did_295, RaDIDVar296=[0,1], OffsetDIDVar296=0, ResolDIDVar296=1, DataTypeDIDVar296=uint8, In_DID_Name_296=Val_did_296, RaDIDVar297=[0,1], OffsetDIDVar297=0, ResolDIDVar297=1, DataTypeDIDVar297=uint8, In_DID_Name_297=Val_did_297, RaDIDVar298=[0,1], OffsetDIDVar298=0, ResolDIDVar298=1, DataTypeDIDVar298=uint8, In_DID_Name_298=Val_did_298, RaDIDVar299=[0,1], OffsetDIDVar299=0, ResolDIDVar299=1, DataTypeDIDVar299=uint8, In_DID_Name_299=Val_did_299, RaDIDVar300=[0,1], OffsetDIDVar300=0, ResolDIDVar300=1, DataTypeDIDVar300=uint8, In_DID_Name_300=Val_did_300, RaDIDVar301=[0,1], OffsetDIDVar301=0, ResolDIDVar301=1, DataTypeDIDVar301=uint8, In_DID_Name_301=Val_did_301, RaDIDVar302=[0,1], OffsetDIDVar302=0, ResolDIDVar302=1, DataTypeDIDVar302=uint8, In_DID_Name_302=Val_did_302, RaDIDVar303=[0,1], OffsetDIDVar303=0, ResolDIDVar303=1, DataTypeDIDVar303=uint8, In_DID_Name_303=Val_did_303, RaDIDVar304=[0,1], OffsetDIDVar304=0, ResolDIDVar304=1, DataTypeDIDVar304=uint8, In_DID_Name_304=Val_did_304, RaDIDVar305=[0,1], OffsetDIDVar305=0, ResolDIDVar305=1, DataTypeDIDVar305=uint8, In_DID_Name_305=Val_did_305, RaDIDVar306=[0,1], OffsetDIDVar306=0, ResolDIDVar306=1, DataTypeDIDVar306=uint8, In_DID_Name_306=Val_did_306, RaDIDVar307=[0,1], OffsetDIDVar307=0, ResolDIDVar307=1, DataTypeDIDVar307=uint8, In_DID_Name_307=Val_did_307, RaDIDVar308=[0,1], OffsetDIDVar308=0, ResolDIDVar308=1, DataTypeDIDVar308=uint8, In_DID_Name_308=Val_did_308, RaDIDVar309=[0,1], OffsetDIDVar309=0, ResolDIDVar309=1, DataTypeDIDVar309=uint8, In_DID_Name_309=Val_did_309, RaDIDVar310=[0,1], OffsetDIDVar310=0, ResolDIDVar310=1, DataTypeDIDVar310=uint8, In_DID_Name_310=Val_did_310, RaDIDVar311=[0,1], OffsetDIDVar311=0, ResolDIDVar311=1, DataTypeDIDVar311=uint8, In_DID_Name_311=Val_did_311, RaDIDVar312=[0,1], OffsetDIDVar312=0, ResolDIDVar312=1, DataTypeDIDVar312=uint8, In_DID_Name_312=Val_did_312, RaDIDVar313=[0,1], OffsetDIDVar313=0, ResolDIDVar313=1, DataTypeDIDVar313=uint8, In_DID_Name_313=Val_did_313, RaDIDVar314=[0,1], OffsetDIDVar314=0, ResolDIDVar314=1, DataTypeDIDVar314=uint8, In_DID_Name_314=Val_did_314, RaDIDVar315=[0,1], OffsetDIDVar315=0, ResolDIDVar315=1, DataTypeDIDVar315=uint8, In_DID_Name_315=Val_did_315, RaDIDVar316=[0,1], OffsetDIDVar316=0, ResolDIDVar316=1, DataTypeDIDVar316=uint8, In_DID_Name_316=Val_did_316, RaDIDVar317=[0,1], OffsetDIDVar317=0, ResolDIDVar317=1, DataTypeDIDVar317=uint8, In_DID_Name_317=Val_did_317, RaDIDVar318=[0,1], OffsetDIDVar318=0, ResolDIDVar318=1, DataTypeDIDVar318=uint8, In_DID_Name_318=Val_did_318, RaDIDVar319=[0,1], OffsetDIDVar319=0, ResolDIDVar319=1, DataTypeDIDVar319=uint8, In_DID_Name_319=Val_did_319, RaDIDVar320=[0,1], OffsetDIDVar320=0, ResolDIDVar320=1, DataTypeDIDVar320=uint8, In_DID_Name_320=Val_did_320, RaDIDVar321=[0,1], OffsetDIDVar321=0, ResolDIDVar321=1, DataTypeDIDVar321=uint8, In_DID_Name_321=Val_did_321, RaDIDVar322=[0,1], OffsetDIDVar322=0, ResolDIDVar322=1, DataTypeDIDVar322=uint8, In_DID_Name_322=Val_did_322, RaDIDVar323=[0,1], OffsetDIDVar323=0, ResolDIDVar323=1, DataTypeDIDVar323=uint8, In_DID_Name_323=Val_did_323, RaDIDVar324=[0,1], OffsetDIDVar324=0, ResolDIDVar324=1, DataTypeDIDVar324=uint8, In_DID_Name_324=Val_did_324, RaDIDVar325=[0,1], OffsetDIDVar325=0, ResolDIDVar325=1, DataTypeDIDVar325=uint8, In_DID_Name_325=Val_did_325, RaDIDVar326=[0,1], OffsetDIDVar326=0, ResolDIDVar326=1, DataTypeDIDVar326=uint8, In_DID_Name_326=Val_did_326, RaDIDVar327=[0,1], OffsetDIDVar327=0, ResolDIDVar327=1, DataTypeDIDVar327=uint8, In_DID_Name_327=Val_did_327, RaDIDVar328=[0,1], OffsetDIDVar328=0, ResolDIDVar328=1, DataTypeDIDVar328=uint8, In_DID_Name_328=Val_did_328, RaDIDVar329=[0,1], OffsetDIDVar329=0, ResolDIDVar329=1, DataTypeDIDVar329=uint8, In_DID_Name_329=Val_did_329, RaDIDVar330=[0,1], OffsetDIDVar330=0, ResolDIDVar330=1, DataTypeDIDVar330=uint8, In_DID_Name_330=Val_did_330, RaDIDVar331=[0,1], OffsetDIDVar331=0, ResolDIDVar331=1, DataTypeDIDVar331=uint8, In_DID_Name_331=Val_did_331, RaDIDVar332=[0,1], OffsetDIDVar332=0, ResolDIDVar332=1, DataTypeDIDVar332=uint8, In_DID_Name_332=Val_did_332, RaDIDVar333=[0,1], OffsetDIDVar333=0, ResolDIDVar333=1, DataTypeDIDVar333=uint8, In_DID_Name_333=Val_did_333, RaDIDVar334=[0,1], OffsetDIDVar334=0, ResolDIDVar334=1, DataTypeDIDVar334=uint8, In_DID_Name_334=Val_did_334, RaDIDVar335=[0,1], OffsetDIDVar335=0, ResolDIDVar335=1, DataTypeDIDVar335=uint8, In_DID_Name_335=Val_did_335, RaDIDVar336=[0,1], OffsetDIDVar336=0, ResolDIDVar336=1, DataTypeDIDVar336=uint8, In_DID_Name_336=Val_did_336, RaDIDVar337=[0,1], OffsetDIDVar337=0, ResolDIDVar337=1, DataTypeDIDVar337=uint8, In_DID_Name_337=Val_did_337, RaDIDVar338=[0,1], OffsetDIDVar338=0, ResolDIDVar338=1, DataTypeDIDVar338=uint8, In_DID_Name_338=Val_did_338, RaDIDVar339=[0,1], OffsetDIDVar339=0, ResolDIDVar339=1, DataTypeDIDVar339=uint8, In_DID_Name_339=Val_did_339, RaDIDVar340=[0,1], OffsetDIDVar340=0, ResolDIDVar340=1, DataTypeDIDVar340=uint8, In_DID_Name_340=Val_did_340, RaDIDVar341=[0,1], OffsetDIDVar341=0, ResolDIDVar341=1, DataTypeDIDVar341=uint8, In_DID_Name_341=Val_did_341, RaDIDVar342=[0,1], OffsetDIDVar342=0, ResolDIDVar342=1, DataTypeDIDVar342=uint8, In_DID_Name_342=Val_did_342, RaDIDVar343=[0,1], OffsetDIDVar343=0, ResolDIDVar343=1, DataTypeDIDVar343=uint8, In_DID_Name_343=Val_did_343, RaDIDVar344=[0,1], OffsetDIDVar344=0, ResolDIDVar344=1, DataTypeDIDVar344=uint8, In_DID_Name_344=Val_did_344, RaDIDVar345=[0,1], OffsetDIDVar345=0, ResolDIDVar345=1, DataTypeDIDVar345=uint8, In_DID_Name_345=Val_did_345, RaDIDVar346=[0,1], OffsetDIDVar346=0, ResolDIDVar346=1, DataTypeDIDVar346=uint8, In_DID_Name_346=Val_did_346, RaDIDVar347=[0,1], OffsetDIDVar347=0, ResolDIDVar347=1, DataTypeDIDVar347=uint8, In_DID_Name_347=Val_did_347, RaDIDVar348=[0,1], OffsetDIDVar348=0, ResolDIDVar348=1, DataTypeDIDVar348=uint8, In_DID_Name_348=Val_did_348, RaDIDVar349=[0,1], OffsetDIDVar349=0, ResolDIDVar349=1, DataTypeDIDVar349=uint8, In_DID_Name_349=Val_did_349, RaDIDVar350=[0,1], OffsetDIDVar350=0, ResolDIDVar350=1, DataTypeDIDVar350=uint8, In_DID_Name_350=Val_did_350, RaDIDVar351=[0,1], OffsetDIDVar351=0, ResolDIDVar351=1, DataTypeDIDVar351=uint8, In_DID_Name_351=Val_did_351, RaDIDVar352=[0,1], OffsetDIDVar352=0, ResolDIDVar352=1, DataTypeDIDVar352=uint8, In_DID_Name_352=Val_did_352, RaDIDVar353=[0,1], OffsetDIDVar353=0, ResolDIDVar353=1, DataTypeDIDVar353=uint8, In_DID_Name_353=Val_did_353, RaDIDVar354=[0,1], OffsetDIDVar354=0, ResolDIDVar354=1, DataTypeDIDVar354=uint8, In_DID_Name_354=Val_did_354, RaDIDVar355=[0,1], OffsetDIDVar355=0, ResolDIDVar355=1, DataTypeDIDVar355=uint8, In_DID_Name_355=Val_did_355, RaDIDVar356=[0,1], OffsetDIDVar356=0, ResolDIDVar356=1, DataTypeDIDVar356=uint8, In_DID_Name_356=Val_did_356, RaDIDVar357=[0,1], OffsetDIDVar357=0, ResolDIDVar357=1, DataTypeDIDVar357=uint8, In_DID_Name_357=Val_did_357, RaDIDVar358=[0,1], OffsetDIDVar358=0, ResolDIDVar358=1, DataTypeDIDVar358=uint8, In_DID_Name_358=Val_did_358, RaDIDVar359=[0,1], OffsetDIDVar359=0, ResolDIDVar359=1, DataTypeDIDVar359=uint8, In_DID_Name_359=Val_did_359, RaDIDVar360=[0,1], OffsetDIDVar360=0, ResolDIDVar360=1, DataTypeDIDVar360=uint8, In_DID_Name_360=Val_did_360, RaDIDVar361=[0,1], OffsetDIDVar361=0, ResolDIDVar361=1, DataTypeDIDVar361=uint8, In_DID_Name_361=Val_did_361, RaDIDVar362=[0,1], OffsetDIDVar362=0, ResolDIDVar362=1, DataTypeDIDVar362=uint8, In_DID_Name_362=Val_did_362, RaDIDVar363=[0,1], OffsetDIDVar363=0, ResolDIDVar363=1, DataTypeDIDVar363=uint8, In_DID_Name_363=Val_did_363, RaDIDVar364=[0,1], OffsetDIDVar364=0, ResolDIDVar364=1, DataTypeDIDVar364=uint8, In_DID_Name_364=Val_did_364, RaDIDVar365=[0,1], OffsetDIDVar365=0, ResolDIDVar365=1, DataTypeDIDVar365=uint8, In_DID_Name_365=Val_did_365, RaDIDVar366=[0,1], OffsetDIDVar366=0, ResolDIDVar366=1, DataTypeDIDVar366=uint8, In_DID_Name_366=Val_did_366, RaDIDVar367=[0,1], OffsetDIDVar367=0, ResolDIDVar367=1, DataTypeDIDVar367=uint8, In_DID_Name_367=Val_did_367, RaDIDVar368=[0,1], OffsetDIDVar368=0, ResolDIDVar368=1, DataTypeDIDVar368=uint8, In_DID_Name_368=Val_did_368, RaDIDVar369=[0,1], OffsetDIDVar369=0, ResolDIDVar369=1, DataTypeDIDVar369=uint8, In_DID_Name_369=Val_did_369, RaDIDVar370=[0,1], OffsetDIDVar370=0, ResolDIDVar370=1, DataTypeDIDVar370=uint8, In_DID_Name_370=Val_did_370, RaDIDVar371=[0,1], OffsetDIDVar371=0, ResolDIDVar371=1, DataTypeDIDVar371=uint8, In_DID_Name_371=Val_did_371, RaDIDVar372=[0,1], OffsetDIDVar372=0, ResolDIDVar372=1, DataTypeDIDVar372=uint8, In_DID_Name_372=Val_did_372, RaDIDVar373=[0,1], OffsetDIDVar373=0, ResolDIDVar373=1, DataTypeDIDVar373=uint8, In_DID_Name_373=Val_did_373, RaDIDVar374=[0,1], OffsetDIDVar374=0, ResolDIDVar374=1, DataTypeDIDVar374=uint8, In_DID_Name_374=Val_did_374, RaDIDVar375=[0,1], OffsetDIDVar375=0, ResolDIDVar375=1, DataTypeDIDVar375=uint8, In_DID_Name_375=Val_did_375, RaDIDVar376=[0,1], OffsetDIDVar376=0, ResolDIDVar376=1, DataTypeDIDVar376=uint8, In_DID_Name_376=Val_did_376, RaDIDVar377=[0,1], OffsetDIDVar377=0, ResolDIDVar377=1, DataTypeDIDVar377=uint8, In_DID_Name_377=Val_did_377, RaDIDVar378=[0,1], OffsetDIDVar378=0, ResolDIDVar378=1, DataTypeDIDVar378=uint8, In_DID_Name_378=Val_did_378, RaDIDVar379=[0,1], OffsetDIDVar379=0, ResolDIDVar379=1, DataTypeDIDVar379=uint8, In_DID_Name_379=Val_did_379, RaDIDVar380=[0,1], OffsetDIDVar380=0, ResolDIDVar380=1, DataTypeDIDVar380=uint8, In_DID_Name_380=Val_did_380, RaDIDVar381=[0,1], OffsetDIDVar381=0, ResolDIDVar381=1, DataTypeDIDVar381=uint8, In_DID_Name_381=Val_did_381, RaDIDVar382=[0,1], OffsetDIDVar382=0, ResolDIDVar382=1, DataTypeDIDVar382=uint8, In_DID_Name_382=Val_did_382, RaDIDVar383=[0,1], OffsetDIDVar383=0, ResolDIDVar383=1, DataTypeDIDVar383=uint8, In_DID_Name_383=Val_did_383, RaDIDVar384=[0,1], OffsetDIDVar384=0, ResolDIDVar384=1, DataTypeDIDVar384=uint8, In_DID_Name_384=Val_did_384, RaDIDVar385=[0,1], OffsetDIDVar385=0, ResolDIDVar385=1, DataTypeDIDVar385=uint8, In_DID_Name_385=Val_did_385, RaDIDVar386=[0,1], OffsetDIDVar386=0, ResolDIDVar386=1, DataTypeDIDVar386=uint8, In_DID_Name_386=Val_did_386, RaDIDVar387=[0,1], OffsetDIDVar387=0, ResolDIDVar387=1, DataTypeDIDVar387=uint8, In_DID_Name_387=Val_did_387, RaDIDVar388=[0,1], OffsetDIDVar388=0, ResolDIDVar388=1, DataTypeDIDVar388=uint8, In_DID_Name_388=Val_did_388, RaDIDVar389=[0,1], OffsetDIDVar389=0, ResolDIDVar389=1, DataTypeDIDVar389=uint8, In_DID_Name_389=Val_did_389, RaDIDVar390=[0,1], OffsetDIDVar390=0, ResolDIDVar390=1, DataTypeDIDVar390=uint8, In_DID_Name_390=Val_did_390, RaDIDVar391=[0,1], OffsetDIDVar391=0, ResolDIDVar391=1, DataTypeDIDVar391=uint8, In_DID_Name_391=Val_did_391, RaDIDVar392=[0,1], OffsetDIDVar392=0, ResolDIDVar392=1, DataTypeDIDVar392=uint8, In_DID_Name_392=Val_did_392, RaDIDVar393=[0,1], OffsetDIDVar393=0, ResolDIDVar393=1, DataTypeDIDVar393=uint8, In_DID_Name_393=Val_did_393, RaDIDVar394=[0,1], OffsetDIDVar394=0, ResolDIDVar394=1, DataTypeDIDVar394=uint8, In_DID_Name_394=Val_did_394, RaDIDVar395=[0,1], OffsetDIDVar395=0, ResolDIDVar395=1, DataTypeDIDVar395=uint8, In_DID_Name_395=Val_did_395, RaDIDVar396=[0,1], OffsetDIDVar396=0, ResolDIDVar396=1, DataTypeDIDVar396=uint8, In_DID_Name_396=Val_did_396, RaDIDVar397=[0,1], OffsetDIDVar397=0, ResolDIDVar397=1, DataTypeDIDVar397=uint8, In_DID_Name_397=Val_did_397, RaDIDVar398=[0,1], OffsetDIDVar398=0, ResolDIDVar398=1, DataTypeDIDVar398=uint8, In_DID_Name_398=Val_did_398, RaDIDVar399=[0,1], OffsetDIDVar399=0, ResolDIDVar399=1, DataTypeDIDVar399=uint8, In_DID_Name_399=Val_did_399, RaDIDVar400=[0,1], OffsetDIDVar400=0, ResolDIDVar400=1, DataTypeDIDVar400=uint8, In_DID_Name_400=Val_did_400}
      mask prompts: DIDAbstract "DID Abstract"; NumDIDVar "Number of  DID Variables"; RaDIDVar1 "Range (Min,Max)"; OffsetDIDVar1 "Offset"; ResolDIDVar1 "Resolution"; DataTypeDIDVar1 "DID Data Type"; In_DID_Name_1 "Input DID Name"; RaDIDVar2 "Range (Min,Max)"; OffsetDIDVar2 "Offset"; ResolDIDVar2 "Resolution"; DataTypeDIDVar2 "DID Data Type"; In_DID_Name_2 "Input DID Name"; RaDIDVar3 "Range (Min,Max)"; OffsetDIDVar3 "Offset"; ResolDIDVar3 "Resolution"; DataTypeDIDVar3 "DID Data Type"; In_DID_Name_3 "Input DID Name"; RaDIDVar4 "Range (Min,Max)"; OffsetDIDVar4 "Offset"; ResolDIDVar4 "Resolution"; DataTypeDIDVar4 "DID Data Type"; In_DID_Name_4 "Input DID Name"; RaDIDVar5 "Range (Min,Max)"; OffsetDIDVar5 "Offset"; ResolDIDVar5 "Resolution"; DataTypeDIDVar5 "DID Data Type"; In_DID_Name_5 "Input DID Name"; RaDIDVar6 "Range (Min,Max)"; OffsetDIDVar6 "Offset"; ResolDIDVar6 "Resolution"; DataTypeDIDVar6 "DID Data Type"; In_DID_Name_6 "Input DID Name"; RaDIDVar7 "Range (Min,Max)"; OffsetDIDVar7 "Offset"; ResolDIDVar7 "Resolution"; DataTypeDIDVar7 "DID Data Type"; In_DID_Name_7 "Input DID Name"; RaDIDVar8 "Range (Min,Max)"; OffsetDIDVar8 "Offset"; ResolDIDVar8 "Resolution"; DataTypeDIDVar8 "DID Data Type"; In_DID_Name_8 "Input DID Name"; RaDIDVar9 "Range (Min,Max)"; OffsetDIDVar9 "Offset"; ResolDIDVar9 "Resolution"; DataTypeDIDVar9 "DID Data Type"; In_DID_Name_9 "Input DID Name"; RaDIDVar10 "Range (Min,Max)"; OffsetDIDVar10 "Offset"; ResolDIDVar10 "Resolution"; DataTypeDIDVar10 "DID Data Type"; In_DID_Name_10 "Input DID Name"; RaDIDVar11 "Range (Min,Max)"; OffsetDIDVar11 "Offset"; ResolDIDVar11 "Resolution"; DataTypeDIDVar11 "DID Data Type"; In_DID_Name_11 "Input DID Name"; RaDIDVar12 "Range (Min,Max)"; OffsetDIDVar12 "Offset"; ResolDIDVar12 "Resolution"; DataTypeDIDVar12 "DID Data Type"; In_DID_Name_12 "Input DID Name"; RaDIDVar13 "Range (Min,Max)"; OffsetDIDVar13 "Offset"; ResolDIDVar13 "Resolution"; DataTypeDIDVar13 "DID Data Type"; In_DID_Name_13 "Input DID Name"; RaDIDVar14 "Range (Min,Max)"; OffsetDIDVar14 "Offset"; ResolDIDVar14 "Resolution"; DataTypeDIDVar14 "DID Data Type"; In_DID_Name_14 "Input DID Name"; RaDIDVar15 "Range (Min,Max)"; OffsetDIDVar15 "Offset"; ResolDIDVar15 "Resolution"; DataTypeDIDVar15 "DID Data Type"; In_DID_Name_15 "Input DID Name"; RaDIDVar16 "Range (Min,Max)"; OffsetDIDVar16 "Offset"; ResolDIDVar16 "Resolution"; DataTypeDIDVar16 "DID Data Type"; In_DID_Name_16 "Input DID Name"; RaDIDVar17 "Range (Min,Max)"; OffsetDIDVar17 "Offset"; ResolDIDVar17 "Resolution"; DataTypeDIDVar17 "DID Data Type"; In_DID_Name_17 "Input DID Name"; RaDIDVar18 "Range (Min,Max)"; OffsetDIDVar18 "Offset"; ResolDIDVar18 "Resolution"; DataTypeDIDVar18 "DID Data Type"; In_DID_Name_18 "Input DID Name"; RaDIDVar19 "Range (Min,Max)"; OffsetDIDVar19 "Offset"; ResolDIDVar19 "Resolution"; DataTypeDIDVar19 "DID Data Type"; In_DID_Name_19 "Input DID Name"; RaDIDVar20 "Range (Min,Max)"; OffsetDIDVar20 "Offset"; ResolDIDVar20 "Resolution"; DataTypeDIDVar20 "DID Data Type"; In_DID_Name_20 "Input DID Name"; RaDIDVar21 "Range (Min,Max)"; OffsetDIDVar21 "Offset"; ResolDIDVar21 "Resolution"; DataTypeDIDVar21 "DID Data Type"; In_DID_Name_21 "Input DID Name"; RaDIDVar22 "Range (Min,Max)"; OffsetDIDVar22 "Offset"; ResolDIDVar22 "Resolution"; DataTypeDIDVar22 "DID Data Type"; In_DID_Name_22 "Input DID Name"; RaDIDVar23 "Range (Min,Max)"; OffsetDIDVar23 "Offset"; ResolDIDVar23 "Resolution"; DataTypeDIDVar23 "DID Data Type"; In_DID_Name_23 "Input DID Name"; RaDIDVar24 "Range (Min,Max)"; OffsetDIDVar24 "Offset"; ResolDIDVar24 "Resolution"; DataTypeDIDVar24 "DID Data Type"; In_DID_Name_24 "Input DID Name"; RaDIDVar25 "Range (Min,Max)"; OffsetDIDVar25 "Offset"; ResolDIDVar25 "Resolution"; DataTypeDIDVar25 "DID Data Type"; In_DID_Name_25 "Input DID Name"; RaDIDVar26 "Range (Min,Max)"; OffsetDIDVar26 "Offset"; ResolDIDVar26 "Resolution"; DataTypeDIDVar26 "DID Data Type"; In_DID_Name_26 "Input DID Name"; RaDIDVar27 "Range (Min,Max)"; OffsetDIDVar27 "Offset"; ResolDIDVar27 "Resolution"; DataTypeDIDVar27 "DID Data Type"; In_DID_Name_27 "Input DID Name"; RaDIDVar28 "Range (Min,Max)"; OffsetDIDVar28 "Offset"; ResolDIDVar28 "Resolution"; DataTypeDIDVar28 "DID Data Type"; In_DID_Name_28 "Input DID Name"; RaDIDVar29 "Range (Min,Max)"; OffsetDIDVar29 "Offset"; ResolDIDVar29 "Resolution"; DataTypeDIDVar29 "DID Data Type"; In_DID_Name_29 "Input DID Name"; RaDIDVar30 "Range (Min,Max)"; OffsetDIDVar30 "Offset"; ResolDIDVar30 "Resolution"; DataTypeDIDVar30 "DID Data Type"; In_DID_Name_30 "Input DID Name"; RaDIDVar31 "Range (Min,Max)"; OffsetDIDVar31 "Offset"; ResolDIDVar31 "Resolution"; DataTypeDIDVar31 "DID Data Type"; In_DID_Name_31 "Input DID Name"; RaDIDVar32 "Range (Min,Max)"; OffsetDIDVar32 "Offset"; ResolDIDVar32 "Resolution"; DataTypeDIDVar32 "DID Data Type"; In_DID_Name_32 "Input DID Name"; RaDIDVar33 "Range (Min,Max)"; OffsetDIDVar33 "Offset"; ResolDIDVar33 "Resolution"; DataTypeDIDVar33 "DID Data Type"; In_DID_Name_33 "Input DID Name"; RaDIDVar34 "Range (Min,Max)"; OffsetDIDVar34 "Offset"; ResolDIDVar34 "Resolution"; DataTypeDIDVar34 "DID Data Type"; In_DID_Name_34 "Input DID Name"; RaDIDVar35 "Range (Min,Max)"; OffsetDIDVar35 "Offset"; ResolDIDVar35 "Resolution"; DataTypeDIDVar35 "DID Data Type"; In_DID_Name_35 "Input DID Name"; RaDIDVar36 "Range (Min,Max)"; OffsetDIDVar36 "Offset"; ResolDIDVar36 "Resolution"; DataTypeDIDVar36 "DID Data Type"; In_DID_Name_36 "Input DID Name"; RaDIDVar37 "Range (Min,Max)"; OffsetDIDVar37 "Offset"; ResolDIDVar37 "Resolution"; DataTypeDIDVar37 "DID Data Type"; In_DID_Name_37 "Input DID Name"; RaDIDVar38 "Range (Min,Max)"; OffsetDIDVar38 "Offset"; ResolDIDVar38 "Resolution"; DataTypeDIDVar38 "DID Data Type"; In_DID_Name_38 "Input DID Name"; RaDIDVar39 "Range (Min,Max)"; OffsetDIDVar39 "Offset"; ResolDIDVar39 "Resolution"; DataTypeDIDVar39 "DID Data Type"; In_DID_Name_39 "Input DID Name"; RaDIDVar40 "Range (Min,Max)"; OffsetDIDVar40 "Offset"; ResolDIDVar40 "Resolution"; DataTypeDIDVar40 "DID Data Type"; In_DID_Name_40 "Input DID Name"; RaDIDVar41 "Range (Min,Max)"; OffsetDIDVar41 "Offset"; ResolDIDVar41 "Resolution"; DataTypeDIDVar41 "DID Data Type"; In_DID_Name_41 "Input DID Name"; RaDIDVar42 "Range (Min,Max)"; OffsetDIDVar42 "Offset"; ResolDIDVar42 "Resolution"; DataTypeDIDVar42 "DID Data Type"; In_DID_Name_42 "Input DID Name"; RaDIDVar43 "Range (Min,Max)"; OffsetDIDVar43 "Offset"; ResolDIDVar43 "Resolution"; DataTypeDIDVar43 "DID Data Type"; In_DID_Name_43 "Input DID Name"; RaDIDVar44 "Range (Min,Max)"; OffsetDIDVar44 "Offset"; ResolDIDVar44 "Resolution"; DataTypeDIDVar44 "DID Data Type"; In_DID_Name_44 "Input DID Name"; RaDIDVar45 "Range (Min,Max)"; OffsetDIDVar45 "Offset"; ResolDIDVar45 "Resolution"; DataTypeDIDVar45 "DID Data Type"; In_DID_Name_45 "Input DID Name"; RaDIDVar46 "Range (Min,Max)"; OffsetDIDVar46 "Offset"; ResolDIDVar46 "Resolution"; DataTypeDIDVar46 "DID Data Type"; In_DID_Name_46 "Input DID Name"; RaDIDVar47 "Range (Min,Max)"; OffsetDIDVar47 "Offset"; ResolDIDVar47 "Resolution"; DataTypeDIDVar47 "DID Data Type"; In_DID_Name_47 "Input DID Name"; RaDIDVar48 "Range (Min,Max)"; OffsetDIDVar48 "Offset"; ResolDIDVar48 "Resolution"; DataTypeDIDVar48 "DID Data Type"; In_DID_Name_48 "Input DID Name"; RaDIDVar49 "Range (Min,Max)"; OffsetDIDVar49 "Offset"; ResolDIDVar49 "Resolution"; DataTypeDIDVar49 "DID Data Type"; In_DID_Name_49 "Input DID Name"; RaDIDVar50 "Range (Min,Max)"; OffsetDIDVar50 "Offset"; ResolDIDVar50 "Resolution"; DataTypeDIDVar50 "DID Data Type"; In_DID_Name_50 "Input DID Name"; RaDIDVar51 "Range (Min,Max)"; OffsetDIDVar51 "Offset"; ResolDIDVar51 "Resolution"; DataTypeDIDVar51 "DID Data Type"; In_DID_Name_51 "Input DID Name"; RaDIDVar52 "Range (Min,Max)"; OffsetDIDVar52 "Offset"; ResolDIDVar52 "Resolution"; DataTypeDIDVar52 "DID Data Type"; In_DID_Name_52 "Input DID Name"; RaDIDVar53 "Range (Min,Max)"; OffsetDIDVar53 "Offset"; ResolDIDVar53 "Resolution"; DataTypeDIDVar53 "DID Data Type"; In_DID_Name_53 "Input DID Name"; RaDIDVar54 "Range (Min,Max)"; OffsetDIDVar54 "Offset"; ResolDIDVar54 "Resolution"; DataTypeDIDVar54 "DID Data Type"; In_DID_Name_54 "Input DID Name"; RaDIDVar55 "Range (Min,Max)"; OffsetDIDVar55 "Offset"; ResolDIDVar55 "Resolution"; DataTypeDIDVar55 "DID Data Type"; In_DID_Name_55 "Input DID Name"; RaDIDVar56 "Range (Min,Max)"; OffsetDIDVar56 "Offset"; ResolDIDVar56 "Resolution"; DataTypeDIDVar56 "DID Data Type"; In_DID_Name_56 "Input DID Name"; RaDIDVar57 "Range (Min,Max)"; OffsetDIDVar57 "Offset"; ResolDIDVar57 "Resolution"; DataTypeDIDVar57 "DID Data Type"; In_DID_Name_57 "Input DID Name"; RaDIDVar58 "Range (Min,Max)"; OffsetDIDVar58 "Offset"; ResolDIDVar58 "Resolution"; DataTypeDIDVar58 "DID Data Type"; In_DID_Name_58 "Input DID Name"; RaDIDVar59 "Range (Min,Max)"; OffsetDIDVar59 "Offset"; ResolDIDVar59 "Resolution"; DataTypeDIDVar59 "DID Data Type"; In_DID_Name_59 "Input DID Name"; RaDIDVar60 "Range (Min,Max)"; OffsetDIDVar60 "Offset"; ResolDIDVar60 "Resolution"; DataTypeDIDVar60 "DID Data Type"; In_DID_Name_60 "Input DID Name"; RaDIDVar61 "Range (Min,Max)"; OffsetDIDVar61 "Offset"; ResolDIDVar61 "Resolution"; DataTypeDIDVar61 "DID Data Type"; In_DID_Name_61 "Input DID Name"; RaDIDVar62 "Range (Min,Max)"; OffsetDIDVar62 "Offset"; ResolDIDVar62 "Resolution"; DataTypeDIDVar62 "DID Data Type"; In_DID_Name_62 "Input DID Name"; RaDIDVar63 "Range (Min,Max)"; OffsetDIDVar63 "Offset"; ResolDIDVar63 "Resolution"; DataTypeDIDVar63 "DID Data Type"; In_DID_Name_63 "Input DID Name"; RaDIDVar64 "Range (Min,Max)"; OffsetDIDVar64 "Offset"; ResolDIDVar64 "Resolution"; DataTypeDIDVar64 "DID Data Type"; In_DID_Name_64 "Input DID Name"; RaDIDVar65 "Range (Min,Max)"; OffsetDIDVar65 "Offset"; ResolDIDVar65 "Resolution"; DataTypeDIDVar65 "DID Data Type"; In_DID_Name_65 "Input DID Name"; RaDIDVar66 "Range (Min,Max)"; OffsetDIDVar66 "Offset"; ResolDIDVar66 "Resolution"; DataTypeDIDVar66 "DID Data Type"; In_DID_Name_66 "Input DID Name"; RaDIDVar67 "Range (Min,Max)"; OffsetDIDVar67 "Offset"; ResolDIDVar67 "Resolution"; DataTypeDIDVar67 "DID Data Type"; In_DID_Name_67 "Input DID Name"; RaDIDVar68 "Range (Min,Max)"; OffsetDIDVar68 "Offset"; ResolDIDVar68 "Resolution"; DataTypeDIDVar68 "DID Data Type"; In_DID_Name_68 "Input DID Name"; RaDIDVar69 "Range (Min,Max)"; OffsetDIDVar69 "Offset"; ResolDIDVar69 "Resolution"; DataTypeDIDVar69 "DID Data Type"; In_DID_Name_69 "Input DID Name"; RaDIDVar70 "Range (Min,Max)"; OffsetDIDVar70 "Offset"; ResolDIDVar70 "Resolution"; DataTypeDIDVar70 "DID Data Type"; In_DID_Name_70 "Input DID Name"; RaDIDVar71 "Range (Min,Max)"; OffsetDIDVar71 "Offset"; ResolDIDVar71 "Resolution"; DataTypeDIDVar71 "DID Data Type"; In_DID_Name_71 "Input DID Name"; RaDIDVar72 "Range (Min,Max)"; OffsetDIDVar72 "Offset"; ResolDIDVar72 "Resolution"; DataTypeDIDVar72 "DID Data Type"; In_DID_Name_72 "Input DID Name"; RaDIDVar73 "Range (Min,Max)"; OffsetDIDVar73 "Offset"; ResolDIDVar73 "Resolution"; DataTypeDIDVar73 "DID Data Type"; In_DID_Name_73 "Input DID Name"; RaDIDVar74 "Range (Min,Max)"; OffsetDIDVar74 "Offset"; ResolDIDVar74 "Resolution"; DataTypeDIDVar74 "DID Data Type"; In_DID_Name_74 "Input DID Name"; RaDIDVar75 "Range (Min,Max)"; OffsetDIDVar75 "Offset"; ResolDIDVar75 "Resolution"; DataTypeDIDVar75 "DID Data Type"; In_DID_Name_75 "Input DID Name"; RaDIDVar76 "Range (Min,Max)"; OffsetDIDVar76 "Offset"; ResolDIDVar76 "Resolution"; DataTypeDIDVar76 "DID Data Type"; In_DID_Name_76 "Input DID Name"; RaDIDVar77 "Range (Min,Max)"; OffsetDIDVar77 "Offset"; ResolDIDVar77 "Resolution"; DataTypeDIDVar77 "DID Data Type"; In_DID_Name_77 "Input DID Name"; RaDIDVar78 "Range (Min,Max)"; OffsetDIDVar78 "Offset"; ResolDIDVar78 "Resolution"; DataTypeDIDVar78 "DID Data Type"; In_DID_Name_78 "Input DID Name"; RaDIDVar79 "Range (Min,Max)"; OffsetDIDVar79 "Offset"; ResolDIDVar79 "Resolution"; DataTypeDIDVar79 "DID Data Type"; In_DID_Name_79 "Input DID Name"; RaDIDVar80 "Range (Min,Max)"; OffsetDIDVar80 "Offset"; ResolDIDVar80 "Resolution"; DataTypeDIDVar80 "DID Data Type"; In_DID_Name_80 "Input DID Name"; RaDIDVar81 "Range (Min,Max)"; OffsetDIDVar81 "Offset"; ResolDIDVar81 "Resolution"; DataTypeDIDVar81 "DID Data Type"; In_DID_Name_81 "Input DID Name"; RaDIDVar82 "Range (Min,Max)"; OffsetDIDVar82 "Offset"; ResolDIDVar82 "Resolution"; DataTypeDIDVar82 "DID Data Type"; In_DID_Name_82 "Input DID Name"; RaDIDVar83 "Range (Min,Max)"; OffsetDIDVar83 "Offset"; ResolDIDVar83 "Resolution"; DataTypeDIDVar83 "DID Data Type"; In_DID_Name_83 "Input DID Name"; RaDIDVar84 "Range (Min,Max)"; OffsetDIDVar84 "Offset"; ResolDIDVar84 "Resolution"; DataTypeDIDVar84 "DID Data Type"; In_DID_Name_84 "Input DID Name"; RaDIDVar85 "Range (Min,Max)"; OffsetDIDVar85 "Offset"; ResolDIDVar85 "Resolution"; DataTypeDIDVar85 "DID Data Type"; In_DID_Name_85 "Input DID Name"; RaDIDVar86 "Range (Min,Max)"; OffsetDIDVar86 "Offset"; ResolDIDVar86 "Resolution"; DataTypeDIDVar86 "DID Data Type"; In_DID_Name_86 "Input DID Name"; RaDIDVar87 "Range (Min,Max)"; OffsetDIDVar87 "Offset"; ResolDIDVar87 "Resolution"; DataTypeDIDVar87 "DID Data Type"; In_DID_Name_87 "Input DID Name"; RaDIDVar88 "Range (Min,Max)"; OffsetDIDVar88 "Offset"; ResolDIDVar88 "Resolution"; DataTypeDIDVar88 "DID Data Type"; In_DID_Name_88 "Input DID Name"; RaDIDVar89 "Range (Min,Max)"; OffsetDIDVar89 "Offset"; ResolDIDVar89 "Resolution"; DataTypeDIDVar89 "DID Data Type"; In_DID_Name_89 "Input DID Name"; RaDIDVar90 "Range (Min,Max)"; OffsetDIDVar90 "Offset"; ResolDIDVar90 "Resolution"; DataTypeDIDVar90 "DID Data Type"; In_DID_Name_90 "Input DID Name"; RaDIDVar91 "Range (Min,Max)"; OffsetDIDVar91 "Offset"; ResolDIDVar91 "Resolution"; DataTypeDIDVar91 "DID Data Type"; In_DID_Name_91 "Input DID Name"; RaDIDVar92 "Range (Min,Max)"; OffsetDIDVar92 "Offset"; ResolDIDVar92 "Resolution"; DataTypeDIDVar92 "DID Data Type"; In_DID_Name_92 "Input DID Name"; RaDIDVar93 "Range (Min,Max)"; OffsetDIDVar93 "Offset"; ResolDIDVar93 "Resolution"; DataTypeDIDVar93 "DID Data Type"; In_DID_Name_93 "Input DID Name"; RaDIDVar94 "Range (Min,Max)"; OffsetDIDVar94 "Offset"; ResolDIDVar94 "Resolution"; DataTypeDIDVar94 "DID Data Type"; In_DID_Name_94 "Input DID Name"; RaDIDVar95 "Range (Min,Max)"; OffsetDIDVar95 "Offset"; ResolDIDVar95 "Resolution"; DataTypeDIDVar95 "DID Data Type"; In_DID_Name_95 "Input DID Name"; RaDIDVar96 "Range (Min,Max)"; OffsetDIDVar96 "Offset"; ResolDIDVar96 "Resolution"; DataTypeDIDVar96 "DID Data Type"; In_DID_Name_96 "Input DID Name"; RaDIDVar97 "Range (Min,Max)"; OffsetDIDVar97 "Offset"; ResolDIDVar97 "Resolution"; DataTypeDIDVar97 "DID Data Type"; In_DID_Name_97 "Input DID Name"; RaDIDVar98 "Range (Min,Max)"; OffsetDIDVar98 "Offset"; ResolDIDVar98 "Resolution"; DataTypeDIDVar98 "DID Data Type"; In_DID_Name_98 "Input DID Name"; RaDIDVar99 "Range (Min,Max)"; OffsetDIDVar99 "Offset"; ResolDIDVar99 "Resolution"; DataTypeDIDVar99 "DID Data Type"; In_DID_Name_99 "Input DID Name"; RaDIDVar100 "Range (Min,Max)"; OffsetDIDVar100 "Offset"; ResolDIDVar100 "Resolution"; DataTypeDIDVar100 "DID Data Type"; In_DID_Name_100 "Input DID Name"; RaDIDVar101 "Range (Min,Max)"; OffsetDIDVar101 "Offset"; ResolDIDVar101 "Resolution"; DataTypeDIDVar101 "DID Data Type"; In_DID_Name_101 "Input DID Name"; RaDIDVar102 "Range (Min,Max)"; OffsetDIDVar102 "Offset"; ResolDIDVar102 "Resolution"; DataTypeDIDVar102 "DID Data Type"; In_DID_Name_102 "Input DID Name"; RaDIDVar103 "Range (Min,Max)"; OffsetDIDVar103 "Offset"; ResolDIDVar103 "Resolution"; DataTypeDIDVar103 "DID Data Type"; In_DID_Name_103 "Input DID Name"; RaDIDVar104 "Range (Min,Max)"; OffsetDIDVar104 "Offset"; ResolDIDVar104 "Resolution"; DataTypeDIDVar104 "DID Data Type"; In_DID_Name_104 "Input DID Name"; RaDIDVar105 "Range (Min,Max)"; OffsetDIDVar105 "Offset"; ResolDIDVar105 "Resolution"; DataTypeDIDVar105 "DID Data Type"; In_DID_Name_105 "Input DID Name"; RaDIDVar106 "Range (Min,Max)"; OffsetDIDVar106 "Offset"; ResolDIDVar106 "Resolution"; DataTypeDIDVar106 "DID Data Type"; In_DID_Name_106 "Input DID Name"; RaDIDVar107 "Range (Min,Max)"; OffsetDIDVar107 "Offset"; ResolDIDVar107 "Resolution"; DataTypeDIDVar107 "DID Data Type"; In_DID_Name_107 "Input DID Name"; RaDIDVar108 "Range (Min,Max)"; OffsetDIDVar108 "Offset"; ResolDIDVar108 "Resolution"; DataTypeDIDVar108 "DID Data Type"; In_DID_Name_108 "Input DID Name"; RaDIDVar109 "Range (Min,Max)"; OffsetDIDVar109 "Offset"; ResolDIDVar109 "Resolution"; DataTypeDIDVar109 "DID Data Type"; In_DID_Name_109 "Input DID Name"; RaDIDVar110 "Range (Min,Max)"; OffsetDIDVar110 "Offset"; ResolDIDVar110 "Resolution"; DataTypeDIDVar110 "DID Data Type"; In_DID_Name_110 "Input DID Name"; RaDIDVar111 "Range (Min,Max)"; OffsetDIDVar111 "Offset"; ResolDIDVar111 "Resolution"; DataTypeDIDVar111 "DID Data Type"; In_DID_Name_111 "Input DID Name"; RaDIDVar112 "Range (Min,Max)"; OffsetDIDVar112 "Offset"; ResolDIDVar112 "Resolution"; DataTypeDIDVar112 "DID Data Type"; In_DID_Name_112 "Input DID Name"; RaDIDVar113 "Range (Min,Max)"; OffsetDIDVar113 "Offset"; ResolDIDVar113 "Resolution"; DataTypeDIDVar113 "DID Data Type"; In_DID_Name_113 "Input DID Name"; RaDIDVar114 "Range (Min,Max)"; OffsetDIDVar114 "Offset"; ResolDIDVar114 "Resolution"; DataTypeDIDVar114 "DID Data Type"; In_DID_Name_114 "Input DID Name"; RaDIDVar115 "Range (Min,Max)"; OffsetDIDVar115 "Offset"; ResolDIDVar115 "Resolution"; DataTypeDIDVar115 "DID Data Type"; In_DID_Name_115 "Input DID Name"; RaDIDVar116 "Range (Min,Max)"; OffsetDIDVar116 "Offset"; ResolDIDVar116 "Resolution"; DataTypeDIDVar116 "DID Data Type"; In_DID_Name_116 "Input DID Name"; RaDIDVar117 "Range (Min,Max)"; OffsetDIDVar117 "Offset"; ResolDIDVar117 "Resolution"; DataTypeDIDVar117 "DID Data Type"; In_DID_Name_117 "Input DID Name"; RaDIDVar118 "Range (Min,Max)"; OffsetDIDVar118 "Offset"; ResolDIDVar118 "Resolution"; DataTypeDIDVar118 "DID Data Type"; In_DID_Name_118 "Input DID Name"; RaDIDVar119 "Range (Min,Max)"; OffsetDIDVar119 "Offset"; ResolDIDVar119 "Resolution"; DataTypeDIDVar119 "DID Data Type"; In_DID_Name_119 "Input DID Name"; RaDIDVar120 "Range (Min,Max)"; OffsetDIDVar120 "Offset"; ResolDIDVar120 "Resolution"; DataTypeDIDVar120 "DID Data Type"; In_DID_Name_120 "Input DID Name"; RaDIDVar121 "Range (Min,Max)"; OffsetDIDVar121 "Offset"; ResolDIDVar121 "Resolution"; DataTypeDIDVar121 "DID Data Type"; In_DID_Name_121 "Input DID Name"; RaDIDVar122 "Range (Min,Max)"; OffsetDIDVar122 "Offset"; ResolDIDVar122 "Resolution"; DataTypeDIDVar122 "DID Data Type"; In_DID_Name_122 "Input DID Name"; RaDIDVar123 "Range (Min,Max)"; OffsetDIDVar123 "Offset"; ResolDIDVar123 "Resolution"; DataTypeDIDVar123 "DID Data Type"; In_DID_Name_123 "Input DID Name"; RaDIDVar124 "Range (Min,Max)"; OffsetDIDVar124 "Offset"; ResolDIDVar124 "Resolution"; DataTypeDIDVar124 "DID Data Type"; In_DID_Name_124 "Input DID Name"; RaDIDVar125 "Range (Min,Max)"; OffsetDIDVar125 "Offset"; ResolDIDVar125 "Resolution"; DataTypeDIDVar125 "DID Data Type"; In_DID_Name_125 "Input DID Name"; RaDIDVar126 "Range (Min,Max)"; OffsetDIDVar126 "Offset"; ResolDIDVar126 "Resolution"; DataTypeDIDVar126 "DID Data Type"; In_DID_Name_126 "Input DID Name"; RaDIDVar127 "Range (Min,Max)"; OffsetDIDVar127 "Offset"; ResolDIDVar127 "Resolution"; DataTypeDIDVar127 "DID Data Type"; In_DID_Name_127 "Input DID Name"; RaDIDVar128 "Range (Min,Max)"; OffsetDIDVar128 "Offset"; ResolDIDVar128 "Resolution"; DataTypeDIDVar128 "DID Data Type"; In_DID_Name_128 "Input DID Name"; RaDIDVar129 "Range (Min,Max)"; OffsetDIDVar129 "Offset"; ResolDIDVar129 "Resolution"; DataTypeDIDVar129 "DID Data Type"; In_DID_Name_129 "Input DID Name"; RaDIDVar130 "Range (Min,Max)"; OffsetDIDVar130 "Offset"; ResolDIDVar130 "Resolution"; DataTypeDIDVar130 "DID Data Type"; In_DID_Name_130 "Input DID Name"; RaDIDVar131 "Range (Min,Max)"; OffsetDIDVar131 "Offset"; ResolDIDVar131 "Resolution"; DataTypeDIDVar131 "DID Data Type"; In_DID_Name_131 "Input DID Name"; RaDIDVar132 "Range (Min,Max)"; OffsetDIDVar132 "Offset"; ResolDIDVar132 "Resolution"; DataTypeDIDVar132 "DID Data Type"; In_DID_Name_132 "Input DID Name"; RaDIDVar133 "Range (Min,Max)"; OffsetDIDVar133 "Offset"; ResolDIDVar133 "Resolution"; DataTypeDIDVar133 "DID Data Type"; In_DID_Name_133 "Input DID Name"; RaDIDVar134 "Range (Min,Max)"; OffsetDIDVar134 "Offset"; ResolDIDVar134 "Resolution"; DataTypeDIDVar134 "DID Data Type"; In_DID_Name_134 "Input DID Name"; RaDIDVar135 "Range (Min,Max)"; OffsetDIDVar135 "Offset"; ResolDIDVar135 "Resolution"; DataTypeDIDVar135 "DID Data Type"; In_DID_Name_135 "Input DID Name"; RaDIDVar136 "Range (Min,Max)"; OffsetDIDVar136 "Offset"; ResolDIDVar136 "Resolution"; DataTypeDIDVar136 "DID Data Type"; In_DID_Name_136 "Input DID Name"; RaDIDVar137 "Range (Min,Max)"; OffsetDIDVar137 "Offset"; ResolDIDVar137 "Resolution"; DataTypeDIDVar137 "DID Data Type"; In_DID_Name_137 "Input DID Name"; RaDIDVar138 "Range (Min,Max)"; OffsetDIDVar138 "Offset"; ResolDIDVar138 "Resolution"; DataTypeDIDVar138 "DID Data Type"; In_DID_Name_138 "Input DID Name"; RaDIDVar139 "Range (Min,Max)"; OffsetDIDVar139 "Offset"; ResolDIDVar139 "Resolution"; DataTypeDIDVar139 "DID Data Type"; In_DID_Name_139 "Input DID Name"; RaDIDVar140 "Range (Min,Max)"; OffsetDIDVar140 "Offset"; ResolDIDVar140 "Resolution"; DataTypeDIDVar140 "DID Data Type"; In_DID_Name_140 "Input DID Name"; RaDIDVar141 "Range (Min,Max)"; OffsetDIDVar141 "Offset"; ResolDIDVar141 "Resolution"; DataTypeDIDVar141 "DID Data Type"; In_DID_Name_141 "Input DID Name"; RaDIDVar142 "Range (Min,Max)"; OffsetDIDVar142 "Offset"; ResolDIDVar142 "Resolution"; DataTypeDIDVar142 "DID Data Type"; In_DID_Name_142 "Input DID Name"; RaDIDVar143 "Range (Min,Max)"; OffsetDIDVar143 "Offset"; ResolDIDVar143 "Resolution"; DataTypeDIDVar143 "DID Data Type"; In_DID_Name_143 "Input DID Name"; RaDIDVar144 "Range (Min,Max)"; OffsetDIDVar144 "Offset"; ResolDIDVar144 "Resolution"; DataTypeDIDVar144 "DID Data Type"; In_DID_Name_144 "Input DID Name"; RaDIDVar145 "Range (Min,Max)"; OffsetDIDVar145 "Offset"; ResolDIDVar145 "Resolution"; DataTypeDIDVar145 "DID Data Type"; In_DID_Name_145 "Input DID Name"; RaDIDVar146 "Range (Min,Max)"; OffsetDIDVar146 "Offset"; ResolDIDVar146 "Resolution"; DataTypeDIDVar146 "DID Data Type"; In_DID_Name_146 "Input DID Name"; RaDIDVar147 "Range (Min,Max)"; OffsetDIDVar147 "Offset"; ResolDIDVar147 "Resolution"; DataTypeDIDVar147 "DID Data Type"; In_DID_Name_147 "Input DID Name"; RaDIDVar148 "Range (Min,Max)"; OffsetDIDVar148 "Offset"; ResolDIDVar148 "Resolution"; DataTypeDIDVar148 "DID Data Type"; In_DID_Name_148 "Input DID Name"; RaDIDVar149 "Range (Min,Max)"; OffsetDIDVar149 "Offset"; ResolDIDVar149 "Resolution"; DataTypeDIDVar149 "DID Data Type"; In_DID_Name_149 "Input DID Name"; RaDIDVar150 "Range (Min,Max)"; OffsetDIDVar150 "Offset"; ResolDIDVar150 "Resolution"; DataTypeDIDVar150 "DID Data Type"; In_DID_Name_150 "Input DID Name"; RaDIDVar151 "Range"; OffsetDIDVar151 "Offset"; ResolDIDVar151 "Resolution"; DataTypeDIDVar151 "DID Data Type"; In_DID_Name_151 "Input DID Name"; RaDIDVar152 "Range (Min,Max)"; OffsetDIDVar152 "Offset"; ResolDIDVar152 "Resolution"; DataTypeDIDVar152 "DID Data Type"; In_DID_Name_152 "Input DID Name"; RaDIDVar153 "Range (Min,Max)"; OffsetDIDVar153 "Offset"; ResolDIDVar153 "Resolution"; DataTypeDIDVar153 "DID Data Type"; In_DID_Name_153 "Input DID Name"; RaDIDVar154 "Range (Min,Max)"; OffsetDIDVar154 "Offset"; ResolDIDVar154 "Resolution"; DataTypeDIDVar154 "DID Data Type"; In_DID_Name_154 "Input DID Name"; RaDIDVar155 "Range (Min,Max)"; OffsetDIDVar155 "Offset"; ResolDIDVar155 "Resolution"; DataTypeDIDVar155 "DID Data Type"; In_DID_Name_155 "Input DID Name"; RaDIDVar156 "Range (Min,Max)"; OffsetDIDVar156 "Offset"; ResolDIDVar156 "Resolution"; DataTypeDIDVar156 "DID Data Type"; In_DID_Name_156 "Input DID Name"; RaDIDVar157 "Range (Min,Max)"; OffsetDIDVar157 "Offset"; ResolDIDVar157 "Resolution"; DataTypeDIDVar157 "DID Data Type"; In_DID_Name_157 "Input DID Name"; RaDIDVar158 "Range (Min,Max)"; OffsetDIDVar158 "Offset"; ResolDIDVar158 "Resolution"; DataTypeDIDVar158 "DID Data Type"; In_DID_Name_158 "Input DID Name"; RaDIDVar159 "Range (Min,Max)"; OffsetDIDVar159 "Offset"; ResolDIDVar159 "Resolution"; DataTypeDIDVar159 "DID Data Type"; In_DID_Name_159 "Input DID Name"; RaDIDVar160 "Range (Min,Max)"; OffsetDIDVar160 "Offset"; ResolDIDVar160 "Resolution"; DataTypeDIDVar160 "DID Data Type"; In_DID_Name_160 "Input DID Name"; RaDIDVar161 "Range (Min,Max)"; OffsetDIDVar161 "Offset"; ResolDIDVar161 "Resolution"; DataTypeDIDVar161 "DID Data Type"; In_DID_Name_161 "Input DID Name"; RaDIDVar162 "Range (Min,Max)"; OffsetDIDVar162 "Offset"; ResolDIDVar162 "Resolution"; DataTypeDIDVar162 "DID Data Type"; In_DID_Name_162 "Input DID Name"; RaDIDVar163 "Range (Min,Max)"; OffsetDIDVar163 "Offset"; ResolDIDVar163 "Resolution"; DataTypeDIDVar163 "DID Data Type"; In_DID_Name_163 "Input DID Name"; RaDIDVar164 "Range (Min,Max)"; OffsetDIDVar164 "Offset"; ResolDIDVar164 "Resolution"; DataTypeDIDVar164 "DID Data Type"; In_DID_Name_164 "Input DID Name"; RaDIDVar165 "Range (Min,Max)"; OffsetDIDVar165 "Offset"; ResolDIDVar165 "Resolution"; DataTypeDIDVar165 "DID Data Type"; In_DID_Name_165 "Input DID Name"; RaDIDVar166 "Range (Min,Max)"; OffsetDIDVar166 "Offset"; ResolDIDVar166 "Resolution"; DataTypeDIDVar166 "DID Data Type"; In_DID_Name_166 "Input DID Name"; RaDIDVar167 "Range (Min,Max)"; OffsetDIDVar167 "Offset"; ResolDIDVar167 "Resolution"; DataTypeDIDVar167 "DID Data Type"; In_DID_Name_167 "Input DID Name"; RaDIDVar168 "Range (Min,Max)"; OffsetDIDVar168 "Offset"; ResolDIDVar168 "Resolution"; DataTypeDIDVar168 "DID Data Type"; In_DID_Name_168 "Input DID Name"; RaDIDVar169 "Range (Min,Max)"; OffsetDIDVar169 "Offset"; ResolDIDVar169 "Resolution"; DataTypeDIDVar169 "DID Data Type"; In_DID_Name_169 "Input DID Name"; RaDIDVar170 "Range (Min,Max)"; OffsetDIDVar170 "Offset"; ResolDIDVar170 "Resolution"; DataTypeDIDVar170 "DID Data Type"; In_DID_Name_170 "Input DID Name"; RaDIDVar171 "Range (Min,Max)"; OffsetDIDVar171 "Offset"; ResolDIDVar171 "Resolution"; DataTypeDIDVar171 "DID Data Type"; In_DID_Name_171 "Input DID Name"; RaDIDVar172 "Range (Min,Max)"; OffsetDIDVar172 "Offset"; ResolDIDVar172 "Resolution"; DataTypeDIDVar172 "DID Data Type"; In_DID_Name_172 "Input DID Name"; RaDIDVar173 "Range (Min,Max)"; OffsetDIDVar173 "Offset"; ResolDIDVar173 "Resolution"; DataTypeDIDVar173 "DID Data Type"; In_DID_Name_173 "Input DID Name"; RaDIDVar174 "Range (Min,Max)"; OffsetDIDVar174 "Offset"; ResolDIDVar174 "Resolution"; DataTypeDIDVar174 "DID Data Type"; In_DID_Name_174 "Input DID Name"; RaDIDVar175 "Range (Min,Max)"; OffsetDIDVar175 "Offset"; ResolDIDVar175 "Resolution"; DataTypeDIDVar175 "DID Data Type"; In_DID_Name_175 "Input DID Name"; RaDIDVar176 "Range (Min,Max)"; OffsetDIDVar176 "Offset"; ResolDIDVar176 "Resolution"; DataTypeDIDVar176 "DID Data Type"; In_DID_Name_176 "Input DID Name"; RaDIDVar177 "Range (Min,Max)"; OffsetDIDVar177 "Offset"; ResolDIDVar177 "Resolution"; DataTypeDIDVar177 "DID Data Type"; In_DID_Name_177 "Input DID Name"; RaDIDVar178 "Range (Min,Max)"; OffsetDIDVar178 "Offset"; ResolDIDVar178 "Resolution"; DataTypeDIDVar178 "DID Data Type"; In_DID_Name_178 "Input DID Name"; RaDIDVar179 "Range (Min,Max)"; OffsetDIDVar179 "Offset"; ResolDIDVar179 "Resolution"; DataTypeDIDVar179 "DID Data Type"; In_DID_Name_179 "Input DID Name"; RaDIDVar180 "Range (Min,Max)"; OffsetDIDVar180 "Offset"; ResolDIDVar180 "Resolution"; DataTypeDIDVar180 "DID Data Type"; In_DID_Name_180 "Input DID Name"; RaDIDVar181 "Range (Min,Max)"; OffsetDIDVar181 "Offset"; ResolDIDVar181 "Resolution"; DataTypeDIDVar181 "DID Data Type"; In_DID_Name_181 "Input DID Name"; RaDIDVar182 "Range (Min,Max)"; OffsetDIDVar182 "Offset"; ResolDIDVar182 "Resolution"; DataTypeDIDVar182 "DID Data Type"; In_DID_Name_182 "Input DID Name"; RaDIDVar183 "Range (Min,Max)"; OffsetDIDVar183 "Offset"; ResolDIDVar183 "Resolution"; DataTypeDIDVar183 "DID Data Type"; In_DID_Name_183 "Input DID Name"; RaDIDVar184 "Range (Min,Max)"; OffsetDIDVar184 "Offset"; ResolDIDVar184 "Resolution"; DataTypeDIDVar184 "DID Data Type"; In_DID_Name_184 "Input DID Name"; RaDIDVar185 "Range (Min,Max)"; OffsetDIDVar185 "Offset"; ResolDIDVar185 "Resolution"; DataTypeDIDVar185 "DID Data Type"; In_DID_Name_185 "Input DID Name"; RaDIDVar186 "Range (Min,Max)"; OffsetDIDVar186 "Offset"; ResolDIDVar186 "Resolution"; DataTypeDIDVar186 "DID Data Type"; In_DID_Name_186 "Input DID Name"; RaDIDVar187 "Range (Min,Max)"; OffsetDIDVar187 "Offset"; ResolDIDVar187 "Resolution"; DataTypeDIDVar187 "DID Data Type"; In_DID_Name_187 "Input DID Name"; RaDIDVar188 "Range (Min,Max)"; OffsetDIDVar188 "Offset"; ResolDIDVar188 "Resolution"; DataTypeDIDVar188 "DID Data Type"; In_DID_Name_188 "Input DID Name"; RaDIDVar189 "Range (Min,Max)"; OffsetDIDVar189 "Offset"; ResolDIDVar189 "Resolution"; DataTypeDIDVar189 "DID Data Type"; In_DID_Name_189 "Input DID Name"; RaDIDVar190 "Range (Min,Max)"; OffsetDIDVar190 "Offset"; ResolDIDVar190 "Resolution"; DataTypeDIDVar190 "DID Data Type"; In_DID_Name_190 "Input DID Name"; RaDIDVar191 "Range (Min,Max)"; OffsetDIDVar191 "Offset"; ResolDIDVar191 "Resolution"; DataTypeDIDVar191 "DID Data Type"; In_DID_Name_191 "Input DID Name"; RaDIDVar192 "Range (Min,Max)"; OffsetDIDVar192 "Offset"; ResolDIDVar192 "Resolution"; DataTypeDIDVar192 "DID Data Type"; In_DID_Name_192 "Input DID Name"; RaDIDVar193 "Range (Min,Max)"; OffsetDIDVar193 "Offset"; ResolDIDVar193 "Resolution"; DataTypeDIDVar193 "DID Data Type"; In_DID_Name_193 "Input DID Name"; RaDIDVar194 "Range (Min,Max)"; OffsetDIDVar194 "Offset"; ResolDIDVar194 "Resolution"; DataTypeDIDVar194 "DID Data Type"; In_DID_Name_194 "Input DID Name"; RaDIDVar195 "Range (Min,Max)"; OffsetDIDVar195 "Offset"; ResolDIDVar195 "Resolution"; DataTypeDIDVar195 "DID Data Type"; In_DID_Name_195 "Input DID Name"; RaDIDVar196 "Range (Min,Max)"; OffsetDIDVar196 "Offset"; ResolDIDVar196 "Resolution"; DataTypeDIDVar196 "DID Data Type"; In_DID_Name_196 "Input DID Name"; RaDIDVar197 "Range (Min,Max)"; OffsetDIDVar197 "Offset"; ResolDIDVar197 "Resolution"; DataTypeDIDVar197 "DID Data Type"; In_DID_Name_197 "Input DID Name"; RaDIDVar198 "Range (Min,Max)"; OffsetDIDVar198 "Offset"; ResolDIDVar198 "Resolution"; DataTypeDIDVar198 "DID Data Type"; In_DID_Name_198 "Input DID Name"; RaDIDVar199 "Range (Min,Max)"; OffsetDIDVar199 "Offset"; ResolDIDVar199 "Resolution"; DataTypeDIDVar199 "DID Data Type"; In_DID_Name_199 "Input DID Name"; RaDIDVar200 "Range (Min,Max)"; OffsetDIDVar200 "Offset"; ResolDIDVar200 "Resolution"; DataTypeDIDVar200 "DID Data Type"; In_DID_Name_200 "Input DID Name"; RaDIDVar201 "Range (Min,Max)"; OffsetDIDVar201 "Offset"; ResolDIDVar201 "Resolution"; DataTypeDIDVar201 "DID Data Type"; In_DID_Name_201 "Input DID Name"; RaDIDVar202 "Range (Min,Max)"; OffsetDIDVar202 "Offset"; ResolDIDVar202 "Resolution"; DataTypeDIDVar202 "DID Data Type"; In_DID_Name_202 "Input DID Name"; RaDIDVar203 "Range (Min,Max)"; OffsetDIDVar203 "Offset"; ResolDIDVar203 "Resolution"; DataTypeDIDVar203 "DID Data Type"; In_DID_Name_203 "Input DID Name"; RaDIDVar204 "Range (Min,Max)"; OffsetDIDVar204 "Offset"; ResolDIDVar204 "Resolution"; DataTypeDIDVar204 "DID Data Type"; In_DID_Name_204 "Input DID Name"; RaDIDVar205 "Range (Min,Max)"; OffsetDIDVar205 "Offset"; ResolDIDVar205 "Resolution"; DataTypeDIDVar205 "DID Data Type"; In_DID_Name_205 "Input DID Name"; RaDIDVar206 "Range (Min,Max)"; OffsetDIDVar206 "Offset"; ResolDIDVar206 "Resolution"; DataTypeDIDVar206 "DID Data Type"; In_DID_Name_206 "Input DID Name"; RaDIDVar207 "Range (Min,Max)"; OffsetDIDVar207 "Offset"; ResolDIDVar207 "Resolution"; DataTypeDIDVar207 "DID Data Type"; In_DID_Name_207 "Input DID Name"; RaDIDVar208 "Range (Min,Max)"; OffsetDIDVar208 "Offset"; ResolDIDVar208 "Resolution"; DataTypeDIDVar208 "DID Data Type"; In_DID_Name_208 "Input DID Name"; RaDIDVar209 "Range (Min,Max)"; OffsetDIDVar209 "Offset"; ResolDIDVar209 "Resolution"; DataTypeDIDVar209 "DID Data Type"; In_DID_Name_209 "Input DID Name"; RaDIDVar210 "Range (Min,Max)"; OffsetDIDVar210 "Offset"; ResolDIDVar210 "Resolution"; DataTypeDIDVar210 "DID Data Type"; In_DID_Name_210 "Input DID Name"; RaDIDVar211 "Range (Min,Max)"; OffsetDIDVar211 "Offset"; ResolDIDVar211 "Resolution"; DataTypeDIDVar211 "DID Data Type"; In_DID_Name_211 "Input DID Name"; RaDIDVar212 "Range (Min,Max)"; OffsetDIDVar212 "Offset"; ResolDIDVar212 "Resolution"; DataTypeDIDVar212 "DID Data Type"; In_DID_Name_212 "Input DID Name"; RaDIDVar213 "Range (Min,Max)"; OffsetDIDVar213 "Offset"; ResolDIDVar213 "Resolution"; DataTypeDIDVar213 "DID Data Type"; In_DID_Name_213 "Input DID Name"; RaDIDVar214 "Range (Min,Max)"; OffsetDIDVar214 "Offset"; ResolDIDVar214 "Resolution"; DataTypeDIDVar214 "DID Data Type"; In_DID_Name_214 "Input DID Name"; RaDIDVar215 "Range (Min,Max)"; OffsetDIDVar215 "Offset"; ResolDIDVar215 "Resolution"; DataTypeDIDVar215 "DID Data Type"; In_DID_Name_215 "Input DID Name"; RaDIDVar216 "Range (Min,Max)"; OffsetDIDVar216 "Offset"; ResolDIDVar216 "Resolution"; DataTypeDIDVar216 "DID Data Type"; In_DID_Name_216 "Input DID Name"; RaDIDVar217 "Range (Min,Max)"; OffsetDIDVar217 "Offset"; ResolDIDVar217 "Resolution"; DataTypeDIDVar217 "DID Data Type"; In_DID_Name_217 "Input DID Name"; RaDIDVar218 "Range (Min,Max)"; OffsetDIDVar218 "Offset"; ResolDIDVar218 "Resolution"; DataTypeDIDVar218 "DID Data Type"; In_DID_Name_218 "Input DID Name"; RaDIDVar219 "Range (Min,Max)"; OffsetDIDVar219 "Offset"; ResolDIDVar219 "Resolution"; DataTypeDIDVar219 "DID Data Type"; In_DID_Name_219 "Input DID Name"; RaDIDVar220 "Range (Min,Max)"; OffsetDIDVar220 "Offset"; ResolDIDVar220 "Resolution"; DataTypeDIDVar220 "DID Data Type"; In_DID_Name_220 "Input DID Name"; RaDIDVar221 "Range (Min,Max)"; OffsetDIDVar221 "Offset"; ResolDIDVar221 "Resolution"; DataTypeDIDVar221 "DID Data Type"; In_DID_Name_221 "Input DID Name"; RaDIDVar222 "Range (Min,Max)"; OffsetDIDVar222 "Offset"; ResolDIDVar222 "Resolution"; DataTypeDIDVar222 "DID Data Type"; In_DID_Name_222 "Input DID Name"; RaDIDVar223 "Range (Min,Max)"; OffsetDIDVar223 "Offset"; ResolDIDVar223 "Resolution"; DataTypeDIDVar223 "DID Data Type"; In_DID_Name_223 "Input DID Name"; RaDIDVar224 "Range (Min,Max)"; OffsetDIDVar224 "Offset"; ResolDIDVar224 "Resolution"; DataTypeDIDVar224 "DID Data Type"; In_DID_Name_224 "Input DID Name"; RaDIDVar225 "Range (Min,Max)"; OffsetDIDVar225 "Offset"; ResolDIDVar225 "Resolution"; DataTypeDIDVar225 "DID Data Type"; In_DID_Name_225 "Input DID Name"; RaDIDVar226 "Range (Min,Max)"; OffsetDIDVar226 "Offset"; ResolDIDVar226 "Resolution"; DataTypeDIDVar226 "DID Data Type"; In_DID_Name_226 "Input DID Name"; RaDIDVar227 "Range (Min,Max)"; OffsetDIDVar227 "Offset"; ResolDIDVar227 "Resolution"; DataTypeDIDVar227 "DID Data Type"; In_DID_Name_227 "Input DID Name"; RaDIDVar228 "Range (Min,Max)"; OffsetDIDVar228 "Offset"; ResolDIDVar228 "Resolution"; DataTypeDIDVar228 "DID Data Type"; In_DID_Name_228 "Input DID Name"; RaDIDVar229 "Range (Min,Max)"; OffsetDIDVar229 "Offset"; ResolDIDVar229 "Resolution"; DataTypeDIDVar229 "DID Data Type"; In_DID_Name_229 "Input DID Name"; RaDIDVar230 "Range (Min,Max)"; OffsetDIDVar230 "Offset"; ResolDIDVar230 "Resolution"; DataTypeDIDVar230 "DID Data Type"; In_DID_Name_230 "Input DID Name"; RaDIDVar231 "Range (Min,Max)"; OffsetDIDVar231 "Offset"; ResolDIDVar231 "Resolution"; DataTypeDIDVar231 "DID Data Type"; In_DID_Name_231 "Input DID Name"; RaDIDVar232 "Range (Min,Max)"; OffsetDIDVar232 "Offset"; ResolDIDVar232 "Resolution"; DataTypeDIDVar232 "DID Data Type"; In_DID_Name_232 "Input DID Name"; RaDIDVar233 "Range (Min,Max)"; OffsetDIDVar233 "Offset"; ResolDIDVar233 "Resolution"; DataTypeDIDVar233 "DID Data Type"; In_DID_Name_233 "Input DID Name"; RaDIDVar234 "Range (Min,Max)"; OffsetDIDVar234 "Offset"; ResolDIDVar234 "Resolution"; DataTypeDIDVar234 "DID Data Type"; In_DID_Name_234 "Input DID Name"; RaDIDVar235 "Range (Min,Max)"; OffsetDIDVar235 "Offset"; ResolDIDVar235 "Resolution"; DataTypeDIDVar235 "DID Data Type"; In_DID_Name_235 "Input DID Name"; RaDIDVar236 "Range (Min,Max)"; OffsetDIDVar236 "Offset"; ResolDIDVar236 "Resolution"; DataTypeDIDVar236 "DID Data Type"; In_DID_Name_236 "Input DID Name"; RaDIDVar237 "Range (Min,Max)"; OffsetDIDVar237 "Offset"; ResolDIDVar237 "Resolution"; DataTypeDIDVar237 "DID Data Type"; In_DID_Name_237 "Input DID Name"; RaDIDVar238 "Range (Min,Max)"; OffsetDIDVar238 "Offset"; ResolDIDVar238 "Resolution"; DataTypeDIDVar238 "DID Data Type"; In_DID_Name_238 "Input DID Name"; RaDIDVar239 "Range (Min,Max)"; OffsetDIDVar239 "Offset"; ResolDIDVar239 "Resolution"; DataTypeDIDVar239 "DID Data Type"; In_DID_Name_239 "Input DID Name"; RaDIDVar240 "Range (Min,Max)"; OffsetDIDVar240 "Offset"; ResolDIDVar240 "Resolution"; DataTypeDIDVar240 "DID Data Type"; In_DID_Name_240 "Input DID Name"; RaDIDVar241 "Range (Min,Max)"; OffsetDIDVar241 "Offset"; ResolDIDVar241 "Resolution"; DataTypeDIDVar241 "DID Data Type"; In_DID_Name_241 "Input DID Name"; RaDIDVar242 "Range (Min,Max)"; OffsetDIDVar242 "Offset"; ResolDIDVar242 "Resolution"; DataTypeDIDVar242 "DID Data Type"; In_DID_Name_242 "Input DID Name"; RaDIDVar243 "Range (Min,Max)"; OffsetDIDVar243 "Offset"; ResolDIDVar243 "Resolution"; DataTypeDIDVar243 "DID Data Type"; In_DID_Name_243 "Input DID Name"; RaDIDVar244 "Range (Min,Max)"; OffsetDIDVar244 "Offset"; ResolDIDVar244 "Resolution"; DataTypeDIDVar244 "DID Data Type"; In_DID_Name_244 "Input DID Name"; RaDIDVar245 "Range (Min,Max)"; OffsetDIDVar245 "Offset"; ResolDIDVar245 "Resolution"; DataTypeDIDVar245 "DID Data Type"; In_DID_Name_245 "Input DID Name"; RaDIDVar246 "Range (Min,Max)"; OffsetDIDVar246 "Offset"; ResolDIDVar246 "Resolution"; DataTypeDIDVar246 "DID Data Type"; In_DID_Name_246 "Input DID Name"; RaDIDVar247 "Range (Min,Max)"; OffsetDIDVar247 "Offset"; ResolDIDVar247 "Resolution"; DataTypeDIDVar247 "DID Data Type"; In_DID_Name_247 "Input DID Name"; RaDIDVar248 "Range (Min,Max)"; OffsetDIDVar248 "Offset"; ResolDIDVar248 "Resolution"; DataTypeDIDVar248 "DID Data Type"; In_DID_Name_248 "Input DID Name"; RaDIDVar249 "Range (Min,Max)"; OffsetDIDVar249 "Offset"; ResolDIDVar249 "Resolution"; DataTypeDIDVar249 "DID Data Type"; In_DID_Name_249 "Input DID Name"; RaDIDVar250 "Range (Min,Max)"; OffsetDIDVar250 "Offset"; ResolDIDVar250 "Resolution"; DataTypeDIDVar250 "DID Data Type"; In_DID_Name_250 "Input DID Name"; RaDIDVar251 "Range (Min,Max)"; OffsetDIDVar251 "Offset"; ResolDIDVar251 "Resolution"; DataTypeDIDVar251 "DID Data Type"; In_DID_Name_251 "Input DID Name"; RaDIDVar252 "Range (Min,Max)"; OffsetDIDVar252 "Offset"; ResolDIDVar252 "Resolution"; DataTypeDIDVar252 "DID Data Type"; In_DID_Name_252 "Input DID Name"; RaDIDVar253 "Range (Min,Max)"; OffsetDIDVar253 "Offset"; ResolDIDVar253 "Resolution"; DataTypeDIDVar253 "DID Data Type"; In_DID_Name_253 "Input DID Name"; RaDIDVar254 "Range (Min,Max)"; OffsetDIDVar254 "Offset"; ResolDIDVar254 "Resolution"; DataTypeDIDVar254 "DID Data Type"; In_DID_Name_254 "Input DID Name"; RaDIDVar255 "Range (Min,Max)"; OffsetDIDVar255 "Offset"; ResolDIDVar255 "Resolution"; DataTypeDIDVar255 "DID Data Type"; In_DID_Name_255 "Input DID Name"; RaDIDVar256 "Range (Min,Max)"; OffsetDIDVar256 "Offset"; ResolDIDVar256 "Resolution"; DataTypeDIDVar256 "DID Data Type"; In_DID_Name_256 "Input DID Name"; RaDIDVar257 "Range (Min,Max)"; OffsetDIDVar257 "Offset"; ResolDIDVar257 "Resolution"; DataTypeDIDVar257 "DID Data Type"; In_DID_Name_257 "Input DID Name"; RaDIDVar258 "Range (Min,Max)"; OffsetDIDVar258 "Offset"; ResolDIDVar258 "Resolution"; DataTypeDIDVar258 "DID Data Type"; In_DID_Name_258 "Input DID Name"; RaDIDVar259 "Range (Min,Max)"; OffsetDIDVar259 "Offset"; ResolDIDVar259 "Resolution"; DataTypeDIDVar259 "DID Data Type"; In_DID_Name_259 "Input DID Name"; RaDIDVar260 "Range (Min,Max)"; OffsetDIDVar260 "Offset"; ResolDIDVar260 "Resolution"; DataTypeDIDVar260 "DID Data Type"; In_DID_Name_260 "Input DID Name"; RaDIDVar261 "Range (Min,Max)"; OffsetDIDVar261 "Offset"; ResolDIDVar261 "Resolution"; DataTypeDIDVar261 "DID Data Type"; In_DID_Name_261 "Input DID Name"; RaDIDVar262 "Range (Min,Max)"; OffsetDIDVar262 "Offset"; ResolDIDVar262 "Resolution"; DataTypeDIDVar262 "DID Data Type"; In_DID_Name_262 "Input DID Name"; RaDIDVar263 "Range (Min,Max)"; OffsetDIDVar263 "Offset"; ResolDIDVar263 "Resolution"; DataTypeDIDVar263 "DID Data Type"; In_DID_Name_263 "Input DID Name"; RaDIDVar264 "Range (Min,Max)"; OffsetDIDVar264 "Offset"; ResolDIDVar264 "Resolution"; DataTypeDIDVar264 "DID Data Type"; In_DID_Name_264 "Input DID Name"; RaDIDVar265 "Range (Min,Max)"; OffsetDIDVar265 "Offset"; ResolDIDVar265 "Resolution"; DataTypeDIDVar265 "DID Data Type"; In_DID_Name_265 "Input DID Name"; RaDIDVar266 "Range (Min,Max)"; OffsetDIDVar266 "Offset"; ResolDIDVar266 "Resolution"; DataTypeDIDVar266 "DID Data Type"; In_DID_Name_266 "Input DID Name"; RaDIDVar267 "Range (Min,Max)"; OffsetDIDVar267 "Offset"; ResolDIDVar267 "Resolution"; DataTypeDIDVar267 "DID Data Type"; In_DID_Name_267 "Input DID Name"; RaDIDVar268 "Range (Min,Max)"; OffsetDIDVar268 "Offset"; ResolDIDVar268 "Resolution"; DataTypeDIDVar268 "DID Data Type"; In_DID_Name_268 "Input DID Name"; RaDIDVar269 "Range (Min,Max)"; OffsetDIDVar269 "Offset"; ResolDIDVar269 "Resolution"; DataTypeDIDVar269 "DID Data Type"; In_DID_Name_269 "Input DID Name"; RaDIDVar270 "Range (Min,Max)"; OffsetDIDVar270 "Offset"; ResolDIDVar270 "Resolution"; DataTypeDIDVar270 "DID Data Type"; In_DID_Name_270 "Input DID Name"; RaDIDVar271 "Range (Min,Max)"; OffsetDIDVar271 "Offset"; ResolDIDVar271 "Resolution"; DataTypeDIDVar271 "DID Data Type"; In_DID_Name_271 "Input DID Name"; RaDIDVar272 "Range (Min,Max)"; OffsetDIDVar272 "Offset"; ResolDIDVar272 "Resolution"; DataTypeDIDVar272 "DID Data Type"; In_DID_Name_272 "Input DID Name"; RaDIDVar273 "Range (Min,Max)"; OffsetDIDVar273 "Offset"; ResolDIDVar273 "Resolution"; DataTypeDIDVar273 "DID Data Type"; In_DID_Name_273 "Input DID Name"; RaDIDVar274 "Range (Min,Max)"; OffsetDIDVar274 "Offset"; ResolDIDVar274 "Resolution"; DataTypeDIDVar274 "DID Data Type"; In_DID_Name_274 "Input DID Name"; RaDIDVar275 "Range (Min,Max)"; OffsetDIDVar275 "Offset"; ResolDIDVar275 "Resolution"; DataTypeDIDVar275 "DID Data Type"; In_DID_Name_275 "Input DID Name"; RaDIDVar276 "Range (Min,Max)"; OffsetDIDVar276 "Offset"; ResolDIDVar276 "Resolution"; DataTypeDIDVar276 "DID Data Type"; In_DID_Name_276 "Input DID Name"; RaDIDVar277 "Range (Min,Max)"; OffsetDIDVar277 "Offset"; ResolDIDVar277 "Resolution"; DataTypeDIDVar277 "DID Data Type"; In_DID_Name_277 "Input DID Name"; RaDIDVar278 "Range (Min,Max)"; OffsetDIDVar278 "Offset"; ResolDIDVar278 "Resolution"; DataTypeDIDVar278 "DID Data Type"; In_DID_Name_278 "Input DID Name"; RaDIDVar279 "Range (Min,Max)"; OffsetDIDVar279 "Offset"; ResolDIDVar279 "Resolution"; DataTypeDIDVar279 "DID Data Type"; In_DID_Name_279 "Input DID Name"; RaDIDVar280 "Range (Min,Max)"; OffsetDIDVar280 "Offset"; ResolDIDVar280 "Resolution"; DataTypeDIDVar280 "DID Data Type"; In_DID_Name_280 "Input DID Name"; RaDIDVar281 "Range (Min,Max)"; OffsetDIDVar281 "Offset"; ResolDIDVar281 "Resolution"; DataTypeDIDVar281 "DID Data Type"; In_DID_Name_281 "Input DID Name"; RaDIDVar282 "Range (Min,Max)"; OffsetDIDVar282 "Offset"; ResolDIDVar282 "Resolution"; DataTypeDIDVar282 "DID Data Type"; In_DID_Name_282 "Input DID Name"; RaDIDVar283 "Range (Min,Max)"; OffsetDIDVar283 "Offset"; ResolDIDVar283 "Resolution"; DataTypeDIDVar283 "DID Data Type"; In_DID_Name_283 "Input DID Name"; RaDIDVar284 "Range (Min,Max)"; OffsetDIDVar284 "Offset"; ResolDIDVar284 "Resolution"; DataTypeDIDVar284 "DID Data Type"; In_DID_Name_284 "Input DID Name"; RaDIDVar285 "Range (Min,Max)"; OffsetDIDVar285 "Offset"; ResolDIDVar285 "Resolution"; DataTypeDIDVar285 "DID Data Type"; In_DID_Name_285 "Input DID Name"; RaDIDVar286 "Range (Min,Max)"; OffsetDIDVar286 "Offset"; ResolDIDVar286 "Resolution"; DataTypeDIDVar286 "DID Data Type"; In_DID_Name_286 "Input DID Name"; RaDIDVar287 "Range (Min,Max)"; OffsetDIDVar287 "Offset"; ResolDIDVar287 "Resolution"; DataTypeDIDVar287 "DID Data Type"; In_DID_Name_287 "Input DID Name"; RaDIDVar288 "Range (Min,Max)"; OffsetDIDVar288 "Offset"; ResolDIDVar288 "Resolution"; DataTypeDIDVar288 "DID Data Type"; In_DID_Name_288 "Input DID Name"; RaDIDVar289 "Range (Min,Max)"; OffsetDIDVar289 "Offset"; ResolDIDVar289 "Resolution"; DataTypeDIDVar289 "DID Data Type"; In_DID_Name_289 "Input DID Name"; RaDIDVar290 "Range (Min,Max)"; OffsetDIDVar290 "Offset"; ResolDIDVar290 "Resolution"; DataTypeDIDVar290 "DID Data Type"; In_DID_Name_290 "Input DID Name"; RaDIDVar291 "Range (Min,Max)"; OffsetDIDVar291 "Offset"; ResolDIDVar291 "Resolution"; DataTypeDIDVar291 "DID Data Type"; In_DID_Name_291 "Input DID Name"; RaDIDVar292 "Range (Min,Max)"; OffsetDIDVar292 "Offset"; ResolDIDVar292 "Resolution"; DataTypeDIDVar292 "DID Data Type"; In_DID_Name_292 "Input DID Name"; RaDIDVar293 "Range (Min,Max)"; OffsetDIDVar293 "Offset"; ResolDIDVar293 "Resolution"; DataTypeDIDVar293 "DID Data Type"; In_DID_Name_293 "Input DID Name"; RaDIDVar294 "Range (Min,Max)"; OffsetDIDVar294 "Offset"; ResolDIDVar294 "Resolution"; DataTypeDIDVar294 "DID Data Type"; In_DID_Name_294 "Input DID Name"; RaDIDVar295 "Range (Min,Max)"; OffsetDIDVar295 "Offset"; ResolDIDVar295 "Resolution"; DataTypeDIDVar295 "DID Data Type"; In_DID_Name_295 "Input DID Name"; RaDIDVar296 "Range (Min,Max)"; OffsetDIDVar296 "Offset"; ResolDIDVar296 "Resolution"; DataTypeDIDVar296 "DID Data Type"; In_DID_Name_296 "Input DID Name"; RaDIDVar297 "Range (Min,Max)"; OffsetDIDVar297 "Offset"; ResolDIDVar297 "Resolution"; DataTypeDIDVar297 "DID Data Type"; In_DID_Name_297 "Input DID Name"; RaDIDVar298 "Range (Min,Max)"; OffsetDIDVar298 "Offset"; ResolDIDVar298 "Resolution"; DataTypeDIDVar298 "DID Data Type"; In_DID_Name_298 "Input DID Name"; RaDIDVar299 "Range (Min,Max)"; OffsetDIDVar299 "Offset"; ResolDIDVar299 "Resolution"; DataTypeDIDVar299 "DID Data Type"; In_DID_Name_299 "Input DID Name"; RaDIDVar300 "Range (Min,Max)"; OffsetDIDVar300 "Offset"; ResolDIDVar300 "Resolution"; DataTypeDIDVar300 "DID Data Type"; In_DID_Name_300 "Input DID Name"; RaDIDVar301 "Range (Min,Max)"; OffsetDIDVar301 "Offset"; ResolDIDVar301 "Resolution"; DataTypeDIDVar301 "DID Data Type"; In_DID_Name_301 "Input DID Name"; RaDIDVar302 "Range (Min,Max)"; OffsetDIDVar302 "Offset"; ResolDIDVar302 "Resolution"; DataTypeDIDVar302 "DID Data Type"; In_DID_Name_302 "Input DID Name"; RaDIDVar303 "Range (Min,Max)"; OffsetDIDVar303 "Offset"; ResolDIDVar303 "Resolution"; DataTypeDIDVar303 "DID Data Type"; In_DID_Name_303 "Input DID Name"; RaDIDVar304 "Range (Min,Max)"; OffsetDIDVar304 "Offset"; ResolDIDVar304 "Resolution"; DataTypeDIDVar304 "DID Data Type"; In_DID_Name_304 "Input DID Name"; RaDIDVar305 "Range (Min,Max)"; OffsetDIDVar305 "Offset"; ResolDIDVar305 "Resolution"; DataTypeDIDVar305 "DID Data Type"; In_DID_Name_305 "Input DID Name"; RaDIDVar306 "Range (Min,Max)"; OffsetDIDVar306 "Offset"; ResolDIDVar306 "Resolution"; DataTypeDIDVar306 "DID Data Type"; In_DID_Name_306 "Input DID Name"; RaDIDVar307 "Range (Min,Max)"; OffsetDIDVar307 "Offset"; ResolDIDVar307 "Resolution"; DataTypeDIDVar307 "DID Data Type"; In_DID_Name_307 "Input DID Name"; RaDIDVar308 "Range (Min,Max)"; OffsetDIDVar308 "Offset"; ResolDIDVar308 "Resolution"; DataTypeDIDVar308 "DID Data Type"; In_DID_Name_308 "Input DID Name"; RaDIDVar309 "Range (Min,Max)"; OffsetDIDVar309 "Offset"; ResolDIDVar309 "Resolution"; DataTypeDIDVar309 "DID Data Type"; In_DID_Name_309 "Input DID Name"; RaDIDVar310 "Range (Min,Max)"; OffsetDIDVar310 "Offset"; ResolDIDVar310 "Resolution"; DataTypeDIDVar310 "DID Data Type"; In_DID_Name_310 "Input DID Name"; RaDIDVar311 "Range (Min,Max)"; OffsetDIDVar311 "Offset"; ResolDIDVar311 "Resolution"; DataTypeDIDVar311 "DID Data Type"; In_DID_Name_311 "Input DID Name"; RaDIDVar312 "Range (Min,Max)"; OffsetDIDVar312 "Offset"; ResolDIDVar312 "Resolution"; DataTypeDIDVar312 "DID Data Type"; In_DID_Name_312 "Input DID Name"; RaDIDVar313 "Range (Min,Max)"; OffsetDIDVar313 "Offset"; ResolDIDVar313 "Resolution"; DataTypeDIDVar313 "DID Data Type"; In_DID_Name_313 "Input DID Name"; RaDIDVar314 "Range (Min,Max)"; OffsetDIDVar314 "Offset"; ResolDIDVar314 "Resolution"; DataTypeDIDVar314 "DID Data Type"; In_DID_Name_314 "Input DID Name"; RaDIDVar315 "Range (Min,Max)"; OffsetDIDVar315 "Offset"; ResolDIDVar315 "Resolution"; DataTypeDIDVar315 "DID Data Type"; In_DID_Name_315 "Input DID Name"; RaDIDVar316 "Range (Min,Max)"; OffsetDIDVar316 "Offset"; ResolDIDVar316 "Resolution"; DataTypeDIDVar316 "DID Data Type"; In_DID_Name_316 "Input DID Name"; RaDIDVar317 "Range (Min,Max)"; OffsetDIDVar317 "Offset"; ResolDIDVar317 "Resolution"; DataTypeDIDVar317 "DID Data Type"; In_DID_Name_317 "Input DID Name"; RaDIDVar318 "Range (Min,Max)"; OffsetDIDVar318 "Offset"; ResolDIDVar318 "Resolution"; DataTypeDIDVar318 "DID Data Type"; In_DID_Name_318 "Input DID Name"; RaDIDVar319 "Range (Min,Max)"; OffsetDIDVar319 "Offset"; ResolDIDVar319 "Resolution"; DataTypeDIDVar319 "DID Data Type"; In_DID_Name_319 "Input DID Name"; RaDIDVar320 "Range (Min,Max)"; OffsetDIDVar320 "Offset"; ResolDIDVar320 "Resolution"; DataTypeDIDVar320 "DID Data Type"; In_DID_Name_320 "Input DID Name"; RaDIDVar321 "Range (Min,Max)"; OffsetDIDVar321 "Offset"; ResolDIDVar321 "Resolution"; DataTypeDIDVar321 "DID Data Type"; In_DID_Name_321 "Input DID Name"; RaDIDVar322 "Range (Min,Max)"; OffsetDIDVar322 "Offset"; ResolDIDVar322 "Resolution"; DataTypeDIDVar322 "DID Data Type"; In_DID_Name_322 "Input DID Name"; RaDIDVar323 "Range (Min,Max)"; OffsetDIDVar323 "Offset"; ResolDIDVar323 "Resolution"; DataTypeDIDVar323 "DID Data Type"; In_DID_Name_323 "Input DID Name"; RaDIDVar324 "Range (Min,Max)"; OffsetDIDVar324 "Offset"; ResolDIDVar324 "Resolution"; DataTypeDIDVar324 "DID Data Type"; In_DID_Name_324 "Input DID Name"; RaDIDVar325 "Range (Min,Max)"; OffsetDIDVar325 "Offset"; ResolDIDVar325 "Resolution"; DataTypeDIDVar325 "DID Data Type"; In_DID_Name_325 "Input DID Name"; RaDIDVar326 "Range (Min,Max)"; OffsetDIDVar326 "Offset"; ResolDIDVar326 "Resolution"; DataTypeDIDVar326 "DID Data Type"; In_DID_Name_326 "Input DID Name"; RaDIDVar327 "Range (Min,Max)"; OffsetDIDVar327 "Offset"; ResolDIDVar327 "Resolution"; DataTypeDIDVar327 "DID Data Type"; In_DID_Name_327 "Input DID Name"; RaDIDVar328 "Range (Min,Max)"; OffsetDIDVar328 "Offset"; ResolDIDVar328 "Resolution"; DataTypeDIDVar328 "DID Data Type"; In_DID_Name_328 "Input DID Name"; RaDIDVar329 "Range (Min,Max)"; OffsetDIDVar329 "Offset"; ResolDIDVar329 "Resolution"; DataTypeDIDVar329 "DID Data Type"; In_DID_Name_329 "Input DID Name"; RaDIDVar330 "Range (Min,Max)"; OffsetDIDVar330 "Offset"; ResolDIDVar330 "Resolution"; DataTypeDIDVar330 "DID Data Type"; In_DID_Name_330 "Input DID Name"; RaDIDVar331 "Range (Min,Max)"; OffsetDIDVar331 "Offset"; ResolDIDVar331 "Resolution"; DataTypeDIDVar331 "DID Data Type"; In_DID_Name_331 "Input DID Name"; RaDIDVar332 "Range (Min,Max)"; OffsetDIDVar332 "Offset"; ResolDIDVar332 "Resolution"; DataTypeDIDVar332 "DID Data Type"; In_DID_Name_332 "Input DID Name"; RaDIDVar333 "Range (Min,Max)"; OffsetDIDVar333 "Offset"; ResolDIDVar333 "Resolution"; DataTypeDIDVar333 "DID Data Type"; In_DID_Name_333 "Input DID Name"; RaDIDVar334 "Range (Min,Max)"; OffsetDIDVar334 "Offset"; ResolDIDVar334 "Resolution"; DataTypeDIDVar334 "DID Data Type"; In_DID_Name_334 "Input DID Name"; RaDIDVar335 "Range (Min,Max)"; OffsetDIDVar335 "Offset"; ResolDIDVar335 "Resolution"; DataTypeDIDVar335 "DID Data Type"; In_DID_Name_335 "Input DID Name"; RaDIDVar336 "Range (Min,Max)"; OffsetDIDVar336 "Offset"; ResolDIDVar336 "Resolution"; DataTypeDIDVar336 "DID Data Type"; In_DID_Name_336 "Input DID Name"; RaDIDVar337 "Range (Min,Max)"; OffsetDIDVar337 "Offset"; ResolDIDVar337 "Resolution"; DataTypeDIDVar337 "DID Data Type"; In_DID_Name_337 "Input DID Name"; RaDIDVar338 "Range (Min,Max)"; OffsetDIDVar338 "Offset"; ResolDIDVar338 "Resolution"; DataTypeDIDVar338 "DID Data Type"; In_DID_Name_338 "Input DID Name"; RaDIDVar339 "Range (Min,Max)"; OffsetDIDVar339 "Offset"; ResolDIDVar339 "Resolution"; DataTypeDIDVar339 "DID Data Type"; In_DID_Name_339 "Input DID Name"; RaDIDVar340 "Range (Min,Max)"; OffsetDIDVar340 "Offset"; ResolDIDVar340 "Resolution"; DataTypeDIDVar340 "DID Data Type"; In_DID_Name_340 "Input DID Name"; RaDIDVar341 "Range (Min,Max)"; OffsetDIDVar341 "Offset"; ResolDIDVar341 "Resolution"; DataTypeDIDVar341 "DID Data Type"; In_DID_Name_341 "Input DID Name"; RaDIDVar342 "Range (Min,Max)"; OffsetDIDVar342 "Offset"; ResolDIDVar342 "Resolution"; DataTypeDIDVar342 "DID Data Type"; In_DID_Name_342 "Input DID Name"; RaDIDVar343 "Range (Min,Max)"; OffsetDIDVar343 "Offset"; ResolDIDVar343 "Resolution"; DataTypeDIDVar343 "DID Data Type"; In_DID_Name_343 "Input DID Name"; RaDIDVar344 "Range (Min,Max)"; OffsetDIDVar344 "Offset"; ResolDIDVar344 "Resolution"; DataTypeDIDVar344 "DID Data Type"; In_DID_Name_344 "Input DID Name"; RaDIDVar345 "Range (Min,Max)"; OffsetDIDVar345 "Offset"; ResolDIDVar345 "Resolution"; DataTypeDIDVar345 "DID Data Type"; In_DID_Name_345 "Input DID Name"; RaDIDVar346 "Range (Min,Max)"; OffsetDIDVar346 "Offset"; ResolDIDVar346 "Resolution"; DataTypeDIDVar346 "DID Data Type"; In_DID_Name_346 "Input DID Name"; RaDIDVar347 "Range (Min,Max)"; OffsetDIDVar347 "Offset"; ResolDIDVar347 "Resolution"; DataTypeDIDVar347 "DID Data Type"; In_DID_Name_347 "Input DID Name"; RaDIDVar348 "Range (Min,Max)"; OffsetDIDVar348 "Offset"; ResolDIDVar348 "Resolution"; DataTypeDIDVar348 "DID Data Type"; In_DID_Name_348 "Input DID Name"; RaDIDVar349 "Range (Min,Max)"; OffsetDIDVar349 "Offset"; ResolDIDVar349 "Resolution"; DataTypeDIDVar349 "DID Data Type"; In_DID_Name_349 "Input DID Name"; RaDIDVar350 "Range (Min,Max)"; OffsetDIDVar350 "Offset"; ResolDIDVar350 "Resolution"; DataTypeDIDVar350 "DID Data Type"; In_DID_Name_350 "Input DID Name"; RaDIDVar351 "Range (Min,Max)"; OffsetDIDVar351 "Offset"; ResolDIDVar351 "Resolution"; DataTypeDIDVar351 "DID Data Type"; In_DID_Name_351 "Input DID Name"; RaDIDVar352 "Range (Min,Max)"; OffsetDIDVar352 "Offset"; ResolDIDVar352 "Resolution"; DataTypeDIDVar352 "DID Data Type"; In_DID_Name_352 "Input DID Name"; RaDIDVar353 "Range (Min,Max)"; OffsetDIDVar353 "Offset"; ResolDIDVar353 "Resolution"; DataTypeDIDVar353 "DID Data Type"; In_DID_Name_353 "Input DID Name"; RaDIDVar354 "Range (Min,Max)"; OffsetDIDVar354 "Offset"; ResolDIDVar354 "Resolution"; DataTypeDIDVar354 "DID Data Type"; In_DID_Name_354 "Input DID Name"; RaDIDVar355 "Range (Min,Max)"; OffsetDIDVar355 "Offset"; ResolDIDVar355 "Resolution"; DataTypeDIDVar355 "DID Data Type"; In_DID_Name_355 "Input DID Name"; RaDIDVar356 "Range (Min,Max)"; OffsetDIDVar356 "Offset"; ResolDIDVar356 "Resolution"; DataTypeDIDVar356 "DID Data Type"; In_DID_Name_356 "Input DID Name"; RaDIDVar357 "Range (Min,Max)"; OffsetDIDVar357 "Offset"; ResolDIDVar357 "Resolution"; DataTypeDIDVar357 "DID Data Type"; In_DID_Name_357 "Input DID Name"; RaDIDVar358 "Range (Min,Max)"; OffsetDIDVar358 "Offset"; ResolDIDVar358 "Resolution"; DataTypeDIDVar358 "DID Data Type"; In_DID_Name_358 "Input DID Name"; RaDIDVar359 "Range (Min,Max)"; OffsetDIDVar359 "Offset"; ResolDIDVar359 "Resolution"; DataTypeDIDVar359 "DID Data Type"; In_DID_Name_359 "Input DID Name"; RaDIDVar360 "Range (Min,Max)"; OffsetDIDVar360 "Offset"; ResolDIDVar360 "Resolution"; DataTypeDIDVar360 "DID Data Type"; In_DID_Name_360 "Input DID Name"; RaDIDVar361 "Range (Min,Max)"; OffsetDIDVar361 "Offset"; ResolDIDVar361 "Resolution"; DataTypeDIDVar361 "DID Data Type"; In_DID_Name_361 "Input DID Name"; RaDIDVar362 "Range (Min,Max)"; OffsetDIDVar362 "Offset"; ResolDIDVar362 "Resolution"; DataTypeDIDVar362 "DID Data Type"; In_DID_Name_362 "Input DID Name"; RaDIDVar363 "Range (Min,Max)"; OffsetDIDVar363 "Offset"; ResolDIDVar363 "Resolution"; DataTypeDIDVar363 "DID Data Type"; In_DID_Name_363 "Input DID Name"; RaDIDVar364 "Range (Min,Max)"; OffsetDIDVar364 "Offset"; ResolDIDVar364 "Resolution"; DataTypeDIDVar364 "DID Data Type"; In_DID_Name_364 "Input DID Name"; RaDIDVar365 "Range (Min,Max)"; OffsetDIDVar365 "Offset"; ResolDIDVar365 "Resolution"; DataTypeDIDVar365 "DID Data Type"; In_DID_Name_365 "Input DID Name"; RaDIDVar366 "Range (Min,Max)"; OffsetDIDVar366 "Offset"; ResolDIDVar366 "Resolution"; DataTypeDIDVar366 "DID Data Type"; In_DID_Name_366 "Input DID Name"; RaDIDVar367 "Range (Min,Max)"; OffsetDIDVar367 "Offset"; ResolDIDVar367 "Resolution"; DataTypeDIDVar367 "DID Data Type"; In_DID_Name_367 "Input DID Name"; RaDIDVar368 "Range (Min,Max)"; OffsetDIDVar368 "Offset"; ResolDIDVar368 "Resolution"; DataTypeDIDVar368 "DID Data Type"; In_DID_Name_368 "Input DID Name"; RaDIDVar369 "Range (Min,Max)"; OffsetDIDVar369 "Offset"; ResolDIDVar369 "Resolution"; DataTypeDIDVar369 "DID Data Type"; In_DID_Name_369 "Input DID Name"; RaDIDVar370 "Range (Min,Max)"; OffsetDIDVar370 "Offset"; ResolDIDVar370 "Resolution"; DataTypeDIDVar370 "DID Data Type"; In_DID_Name_370 "Input DID Name"; RaDIDVar371 "Range (Min,Max)"; OffsetDIDVar371 "Offset"; ResolDIDVar371 "Resolution"; DataTypeDIDVar371 "DID Data Type"; In_DID_Name_371 "Input DID Name"; RaDIDVar372 "Range (Min,Max)"; OffsetDIDVar372 "Offset"; ResolDIDVar372 "Resolution"; DataTypeDIDVar372 "DID Data Type"; In_DID_Name_372 "Input DID Name"; RaDIDVar373 "Range (Min,Max)"; OffsetDIDVar373 "Offset"; ResolDIDVar373 "Resolution"; DataTypeDIDVar373 "DID Data Type"; In_DID_Name_373 "Input DID Name"; RaDIDVar374 "Range (Min,Max)"; OffsetDIDVar374 "Offset"; ResolDIDVar374 "Resolution"; DataTypeDIDVar374 "DID Data Type"; In_DID_Name_374 "Input DID Name"; RaDIDVar375 "Range (Min,Max)"; OffsetDIDVar375 "Offset"; ResolDIDVar375 "Resolution"; DataTypeDIDVar375 "DID Data Type"; In_DID_Name_375 "Input DID Name"; RaDIDVar376 "Range (Min,Max)"; OffsetDIDVar376 "Offset"; ResolDIDVar376 "Resolution"; DataTypeDIDVar376 "DID Data Type"; In_DID_Name_376 "Input DID Name"; RaDIDVar377 "Range (Min,Max)"; OffsetDIDVar377 "Offset"; ResolDIDVar377 "Resolution"; DataTypeDIDVar377 "DID Data Type"; In_DID_Name_377 "Input DID Name"; RaDIDVar378 "Range (Min,Max)"; OffsetDIDVar378 "Offset"; ResolDIDVar378 "Resolution"; DataTypeDIDVar378 "DID Data Type"; In_DID_Name_378 "Input DID Name"; RaDIDVar379 "Range (Min,Max)"; OffsetDIDVar379 "Offset"; ResolDIDVar379 "Resolution"; DataTypeDIDVar379 "DID Data Type"; In_DID_Name_379 "Input DID Name"; RaDIDVar380 "Range (Min,Max)"; OffsetDIDVar380 "Offset"; ResolDIDVar380 "Resolution"; DataTypeDIDVar380 "DID Data Type"; In_DID_Name_380 "Input DID Name"; RaDIDVar381 "Range (Min,Max)"; OffsetDIDVar381 "Offset"; ResolDIDVar381 "Resolution"; DataTypeDIDVar381 "DID Data Type"; In_DID_Name_381 "Input DID Name"; RaDIDVar382 "Range (Min,Max)"; OffsetDIDVar382 "Offset"; ResolDIDVar382 "Resolution"; DataTypeDIDVar382 "DID Data Type"; In_DID_Name_382 "Input DID Name"; RaDIDVar383 "Range (Min,Max)"; OffsetDIDVar383 "Offset"; ResolDIDVar383 "Resolution"; DataTypeDIDVar383 "DID Data Type"; In_DID_Name_383 "Input DID Name"; RaDIDVar384 "Range (Min,Max)"; OffsetDIDVar384 "Offset"; ResolDIDVar384 "Resolution"; DataTypeDIDVar384 "DID Data Type"; In_DID_Name_384 "Input DID Name"; RaDIDVar385 "Range (Min,Max)"; OffsetDIDVar385 "Offset"; ResolDIDVar385 "Resolution"; DataTypeDIDVar385 "DID Data Type"; In_DID_Name_385 "Input DID Name"; RaDIDVar386 "Range (Min,Max)"; OffsetDIDVar386 "Offset"; ResolDIDVar386 "Resolution"; DataTypeDIDVar386 "DID Data Type"; In_DID_Name_386 "Input DID Name"; RaDIDVar387 "Range (Min,Max)"; OffsetDIDVar387 "Offset"; ResolDIDVar387 "Resolution"; DataTypeDIDVar387 "DID Data Type"; In_DID_Name_387 "Input DID Name"; RaDIDVar388 "Range (Min,Max)"; OffsetDIDVar388 "Offset"; ResolDIDVar388 "Resolution"; DataTypeDIDVar388 "DID Data Type"; In_DID_Name_388 "Input DID Name"; RaDIDVar389 "Range (Min,Max)"; OffsetDIDVar389 "Offset"; ResolDIDVar389 "Resolution"; DataTypeDIDVar389 "DID Data Type"; In_DID_Name_389 "Input DID Name"; RaDIDVar390 "Range (Min,Max)"; OffsetDIDVar390 "Offset"; ResolDIDVar390 "Resolution"; DataTypeDIDVar390 "DID Data Type"; In_DID_Name_390 "Input DID Name"; RaDIDVar391 "Range (Min,Max)"; OffsetDIDVar391 "Offset"; ResolDIDVar391 "Resolution"; DataTypeDIDVar391 "DID Data Type"; In_DID_Name_391 "Input DID Name"; RaDIDVar392 "Range (Min,Max)"; OffsetDIDVar392 "Offset"; ResolDIDVar392 "Resolution"; DataTypeDIDVar392 "DID Data Type"; In_DID_Name_392 "Input DID Name"; RaDIDVar393 "Range (Min,Max)"; OffsetDIDVar393 "Offset"; ResolDIDVar393 "Resolution"; DataTypeDIDVar393 "DID Data Type"; In_DID_Name_393 "Input DID Name"; RaDIDVar394 "Range (Min,Max)"; OffsetDIDVar394 "Offset"; ResolDIDVar394 "Resolution"; DataTypeDIDVar394 "DID Data Type"; In_DID_Name_394 "Input DID Name"; RaDIDVar395 "Range (Min,Max)"; OffsetDIDVar395 "Offset"; ResolDIDVar395 "Resolution"; DataTypeDIDVar395 "DID Data Type"; In_DID_Name_395 "Input DID Name"; RaDIDVar396 "Range (Min,Max)"; OffsetDIDVar396 "Offset"; ResolDIDVar396 "Resolution"; DataTypeDIDVar396 "DID Data Type"; In_DID_Name_396 "Input DID Name"; RaDIDVar397 "Range (Min,Max)"; OffsetDIDVar397 "Offset"; ResolDIDVar397 "Resolution"; DataTypeDIDVar397 "DID Data Type"; In_DID_Name_397 "Input DID Name"; RaDIDVar398 "Range (Min,Max)"; OffsetDIDVar398 "Offset"; ResolDIDVar398 "Resolution"; DataTypeDIDVar398 "DID Data Type"; In_DID_Name_398 "Input DID Name"; RaDIDVar399 "Range (Min,Max)"; OffsetDIDVar399 "Offset"; ResolDIDVar399 "Resolution"; DataTypeDIDVar399 "DID Data Type"; In_DID_Name_399 "Input DID Name"; RaDIDVar400 "Range (Min,Max)"; OffsetDIDVar400 "Offset"; ResolDIDVar400 "Resolution"; DataTypeDIDVar400 "DID Data Type"; In_DID_Name_400 "Input DID Name"
      mask help:
      | This function requests to the application a data value of a DID/PID.
      | Reference to AUTOSAR Specification:
      | - AUTOSAR Service Name:  Xxx_ReadData (Ref. [SWS_Dcm_00793])
      |
      | -INPUTS-
      | DID_Variable_[N]: DID Variable No N.
      | -PARAMETERS-
      | DID Abstract: Abstract of DID pre-defined
      | Number of DID Variables: 	Number of DID Variables as input
      | Range of DID Variable [N]: 	Range of DID Variable No N
      | Offset of DID Variable [N]: 	Offset of DID Variable No N
      | Resolution of DID Variable [N]: Resolution of DID Variable No N
      | Size of DID Variable [N]: 	 Number in byte of DID Variable No N
      mask init:
      | libcb=gcb;
      | libh= get_param(libcb,'handle');
      | 
      | %% General declaration
      |    NewStatusstr={};
      |    OldStatusstr={};
      |    flag_convert = 0;
      |    
      | %% Getting bloc general information parameters
      |     DIDAbstractstr=get_param(libcb,'DIDAbstract');
      |     Callbkstr=strcat('DataServices_',strtrim(DIDAbstractstr),'_ReadData');
      |     Data_Value=get(libh,'NumDIDVar'); 
      |     buff_size=0; 
      |     countDID=[];
      | 
      | %% Get and rename with 'DID_Variable_XX' all input under the top subsystem of the library
      |     ini_ip = find_system(libh,'LookUnderMasks','all','FollowLinks','on','SearchDepth','1','BlockType','Inport');
      |     for ip_cnt=1:length(ini_ip)
      |         set(ini_ip(ip_cnt),'Name',['DID_Variable_',num2str(ip_cnt)]);
      |     end
      | 
      |     NumValue=str2double(Data_Value);
      |     countDID=NumValue;
      | 
      | %% Check whether the given configuration is valid or not
      | 
      |     Is_Valid_Config = 1; %By default assume the configration is valid.
      |     for DID_Idx = 1:countDID
      |     Idx = num2str(DID_Idx);
      |     %Get Range (Min, Max)
      |     Range_Of_This_DID = get(libh,['RaDIDVar',Idx]);
      |     Range_Of_This_DID = eval(Range_Of_This_DID);
      |     Phy_Min_Of_This_DID = Range_Of_This_DID(1);
      |     Phy_Max_Of_This_DID = Range_Of_This_DID(2);
      |     %Get Resolution
      |     Res_Of_This_DID = get(libh,['ResolDIDVar',Idx]);
      |     Res_Of_This_DID = eval(Res_Of_This_DID);
      |     %Get Offset
      |     Offset_Of_This_DID = get(libh,['OffsetDIDVar',Idx]);
      |     Offset_Of_This_DID = eval(Offset_Of_This_DID);
      |     %Get Hex_Min_Max as per above config:
      |     Hex_Min = (Phy_Min_Of_This_DID - Offset_Of_This_DID)/Res_Of_This_DID;
      |     Hex_Max = (Phy_Max_Of_This_DID - Offset_Of_This_DID)/Res_Of_This_DID;
      |     DataType_Of_This_DID = get(libh,['DataTypeDIDVar',Idx]);
      |    
      |     switch(DataType_Of_This_DID)
      |         case 'uint8'
      |             if ((Hex_Min < 0) || (Hex_Max > 255) )
      |                 Is_Valid_Config = 0;
      |                 break;
      |             end
      |         case 'uint16'
      |             if ((Hex_Min < 0) || (Hex_Max > 65535) )
      |                 Is_Valid_Config = 0;
      |                 break;
      |             end 
      |         case 'uint32'
      |             if ((Hex_Min < 0) || (Hex_Max > 4294967295) )
      |                 Is_Valid_Config = 0;
      |                 break;
      |             end 
      |         case 'int8'
      |             if ((Hex_Min < -128) || (Hex_Max > 127) )
      |                 Is_Valid_Config = 0;
      |                 break;
      |             end
      |         case 'int16'
      |             if ((Hex_Min < -32768) || (Hex_Max > 32767) )
      |                 Is_Valid_Config = 0;
      |                 break;
      |             end 
      |         case 'int32'
      |             if ((Hex_Min < -2147483648) || (Hex_Max > 2147483647) )
      |                 Is_Valid_Config = 0;
      |                 break;
      |             end 
      |     end    
      |     end
      | 
      |     if ~Is_Valid_Config
      |         errordlg(['Invalid configuration for DID ',num2str(DID_Idx), ' at "',libcb,'"']);
      |         return;
      |     end
      | 
      | %% For each DID variable, we get the new parameters and store it in NewStatusstr
      |     for i=1:NumValue
      |         NewStatusstr{i,1}=str2num(get(libh,['RaDIDVar',num2str(i)]));
      |         NewStatusstr{i,2}=str2num(get(libh,['OffsetDIDVar',num2str(i)]));
      |         NewStatusstr{i,3}=str2num(get(libh,['ResolDIDVar',num2str(i)]));
      |         NewStatusstr{i,4}=str2num(get(libh,['DataTypeDIDVar',num2str(i)]));
      |     end
      | 
      | %% Setting several path of elements
      |     hh = strcat(libcb,'/Conversion_Subsystem');
      |     calbck = strcat(libcb,'/Callback_Subsystem');
      |     trm = strcat(libcb,'/Data');
      |     trmreturntype = strcat(libcb,'/Std_ReturnType');
      | 
      | %% Setting correct position of the Conversion_Subsystem
      |     conv_sub_pos = [];
      |     if NumValue <= 2
      |         conv_sub_pos = [160 48 360 119];
      |     else
      |         conv_sub_pos = [160 48 360 119+((NumValue-2)*35)];
      |     end
      |     set_param(hh,'Position',conv_sub_pos);
      | 
      | %% Setting correct position of the Callback_Subsystem
      |     ph_hh = get_param(hh,'PortHandles');
      |     ph_hh_out_pos = get_param(ph_hh.Outport(1),'Position');
      |     calbck_pos = [470 (ph_hh_out_pos(2)-28)+5 685 (ph_hh_out_pos(2)+28)+5];
      |     set_param(calbck,'Position',calbck_pos);
      | 
      | %% Setting positions of output wires
      |     ph_calbk = get_param(calbck,'PortHandles');
      |     ph_calbk_out_pos = get_param(ph_calbk.Outport(1),'Position');
      |     set_param(trm,'Position',[805 ph_calbk_out_pos(2)-10 825 ph_calbk_out_pos(2)+10]);
      |     ph_calbk_out_pos = get_param(ph_calbk.Outport(2),'Position');
      |     set_param(trmreturntype,'Position',[805 ph_calbk_out_pos(2)-10 825 ph_calbk_out_pos(2)+10]);
      | 
      | %% For each existing AEMS_FLOAT_TO_FXP_WITH_LIMIT_XX, we get its parameters and store it in OldStatusstr
      |     k=get_param(find_system(hh,'FollowLinks','on','LookunderMasks','all','regexp','on','Name','^AEMS_TO_FXP_WITH_LIMIT'),'Name');
      |     for i = 1:size(k,1)
      |         t_fx_fl = [hh,'/AEMS_TO_FXP_WITH_LIMIT_',num2str(i)];
      |         btype = get_param(t_fx_fl,'BlockType');
      |         if strcmp(btype,'DataTypeConversion')
      |             OldStatusstr{i,3} = 1;
      |             OldStatusstr{i,2} = 0;
      |             OldStatusstr{i,1} = [0,1];
      |             OldStatusstr{i,4} = 1;
      |         else
      |             OldStatusstr{i,3}=str2double(get_param(t_fx_fl,'Resol'));
      |             OldStatusstr{i,2}=str2double(get_param(t_fx_fl,'Offset'));
      |             OldStatusstr{i,1}=[str2double(get_param(t_fx_fl,'Min')),str2double(get_param(t_fx_fl,'Max'))];
      |             inblkhandles=get_param(t_fx_fl, 'LineHandles');
      |             OldStatusstr{i,4}=length(get(inblkhandles.Outport,'DstBlockHandle'));
      |         end
      |     end
      | 
      | % buff_size = get_param(gcbh,'BufferSizeinBytes');
      |     k2=find_system(libcb,'SearchDepth',1,'FollowLinks','on','LookunderMasks','all','BlockType','Inport');
      |     k=get_param(k2,'Name');
      | 
      | %% Check if any data was modified and the library block needs update
      |     bModified=0;
      |     if size(NewStatusstr,1)~= size(OldStatusstr,1)
      |         bModified=1;
      |     else
      |         for i=1:size(NewStatusstr,1)
      |             for ii=1:4
      |                 if ~(isequal(OldStatusstr{i,ii},NewStatusstr{i,ii}))
      |                     bModified=1;
      |                     break;
      |                 end
      |             end
      |             if bModified==1
      |                 break;
      |             end
      |         end
      |     end
      | 
      | %% Update the block if any modification is detected
      | if bModified
      |     
      | %% Getting the total number of bytes necessary by adding each "Number of Bytes" field into buff_size
      |     for i=1:NumValue
      |         %buff_size=buff_size+str2double(get(libh,['DataTypeDIDVar',num2str(i)]));
      |         
      |         curDt = get(libh,['DataTypeDIDVar',num2str(i)]);
      |         if(strcmp(curDt, 'int8') || strcmp (curDt, 'uint8'))
      |             buff_size=buff_size+1;
      |         elseif(strcmp(curDt, 'int16') || strcmp (curDt, 'uint16'))
      |             buff_size=buff_size+2;
      |         else
      |             buff_size=buff_size+4;
      |         end
      |     end
      |     
      | 
      | %% Check that the range parameter is a two variable array
      |     for i=1:NumValue
      |         if length(str2double(get(libh,['RaDIDVar',num2str(i)])))~=2
      |             %       error('Range of DID Variables should be an array of [Min,Max]');
      |         end
      |     end
      | 
      | %% Get the position of the outport of the Conversion_Subsystem
      |     blockpath = [hh,'/Value_Read_xxxx_DCM'];
      |     inblkhandles=get_param(blockpath, 'PortHandles');
      |     pos=get_param(inblkhandles.Inport(1),'position');
      |     posport=[50 50]; %get_param(inblkhandles.Outport(1),'position');
      | 
      | %% Delete each line in Conversion_Subsystem apart from the outport one
      |     k2=find_system(hh,'LookUnderMasks', 'all','FindAll', 'on','Type', 'line' );
      |     for j=1:size(k2,1)
      |         try
      |             srchdl=get_param(k2(j),'SrcBlockHandle');
      |             dsthdl=get_param(k2(j),'DstBlockHandle');
      |             if (length(srchdl)~=1||srchdl(1)<0||~strcmpi(get_param(srchdl(1),'BlockType'),'Mux'))...
      |                     &&(length(dsthdl)~=1||dsthdl(1)<0||~strcmpi(get_param(dsthdl(1),'BlockType'),'Outport'))
      |                 delete_line(k2(j));
      |             end
      |         end
      |     end
      | 
      | %% Delete inport and their lines in the top level of the library
      | % buff_size = get_param(gcbh,'BufferSizeinBytes');
      |     k2=find_system(libcb,'SearchDepth',1,'FollowLinks','on','LookunderMasks','all','BlockType','Inport');
      |     for j = 1:length(k2)
      |         if j > NumValue
      |             try
      |                 outp=get_param(k2{j},'LineHandles');
      |                 delete_line(outp.Outport);
      |                 delete_block(k2{j});
      |             end
      |         end
      |     end
      | 
      | %% Delete each inport in Conversion_Subsystem
      | % buff_size = get_param(gcbh,'BufferSizeinBytes');
      |     k2=find_system(hh,'FollowLinks','on','BlockType','Inport');
      | % if size(k,1)~= str2num(buf)
      |     for j = 1:length(k2)
      |         try
      |             if j > NumValue
      |                 delete_block(k2{j});
